simulink model "sim_tcyb_2024_att_ctrl"  (R2020a)
settings: Solver=ode4  StartTime=0.0  StopTime=30.0  FixedStep=0.01  RelTol=1e-3
values from neighbouring files (symbols this model uses):
  c1_diff_sigma_bar_w = diag([12; 12; 12])    [init_tcyb_2024_att_ctrl.m]
  c1_diff_ui = diag([25; 30; 20])    [init_tcyb_2024_att_ctrl.m]
  c2_diff_sigma_bar_w = diag([12; 12; 12])    [init_tcyb_2024_att_ctrl.m]
  c2_diff_ui = diag([50; 50; 10])    [init_tcyb_2024_att_ctrl.m]
  c3_diff_sigma_bar_w = diag([15; 15; 15])    [init_tcyb_2024_att_ctrl.m]
  c3_diff_ui = diag([15; 15; 10])    [init_tcyb_2024_att_ctrl.m]
  dw_aa_t = 0.2 * ones(3, 5) + ( 1.0 - 0.2 ) * rand(3, 5)    [init_tcyb_2024_att_ctrl.m]
  dw_ff_t = [ 0.4 * ones(1, 5) + ( 1.0 - 0.4 ) * rand(1, 5);                      0.4 * ones(1, 5) + ( 1.0 - 0.4 ) * rand(1, 5);                      0.2 * ones(1, 5) + ( 0.6 - 0.2 ) * rand(1, 5) ]    [init_tcyb_2024_att_ctrl.m]
  dw_phi_t = ( - pi / 2 ) * ones(3, 5) + ( pi / 2 - ( - pi / 2 ) ) * rand(3, 5)    [init_tcyb_2024_att_ctrl.m]
  dwci_init = zeros(3,NF)    [init_tcyb_2024_att_ctrl.m]
  h1w = diag([20.0; 20.0; 20.0])    [init_tcyb_2024_att_ctrl.m]
  h2w = diag([30.0; 35.0; 35.0])    [init_tcyb_2024_att_ctrl.m]
  h3w = diag([30.0; 25.0; 30.0])    [init_tcyb_2024_att_ctrl.m]
  Ji = zeros(3,3,NF)    [init_tcyb_2024_att_ctrl.m]
  ksg = diag([10.0, 10.0, 8.0])    [init_tcyb_2024_att_ctrl.m]
  kw = diag([10.0, 10.0, 8.0])    [init_tcyb_2024_att_ctrl.m]
  l1 = diag([5.0, 5.0, 4.0])    [init_tcyb_2024_att_ctrl.m]
  l2 = diag([5.0, 5.0, 4.0])    [init_tcyb_2024_att_ctrl.m]
  Lamd_diff_sigma_bar_w = 0.8    [init_tcyb_2024_att_ctrl.m]
  Lamd_diff_ui = 0.8    [init_tcyb_2024_att_ctrl.m]
  mu = diag([10.0, 10.0, 10.0, 8.0, 8.0, 8.0])    [init_tcyb_2024_att_ctrl.m]
  mu_d_w = 100    [init_tcyb_2024_att_ctrl.m]
  pos0 = zeros(3, 1)    [init_tcyb_2024_att_ctrl.m]
  PZ0 = P0(3)    [init_tcyb_2024_att_ctrl.m]
  PZ1 = 10    [init_tcyb_2024_att_ctrl.m]
  R0 = 4    [init_tcyb_2024_att_ctrl.m]
  R1 = 8    [init_tcyb_2024_att_ctrl.m]
  Rei_init = zeros(3,3,NF)    [init_tcyb_2024_att_ctrl.m]
  Ri_init = zeros(3,3,NF)    [init_tcyb_2024_att_ctrl.m]
  Rx2 = 10    [init_tcyb_2024_att_ctrl.m]
  Ry2 = 6    [init_tcyb_2024_att_ctrl.m]
  Rz2 = 4    [init_tcyb_2024_att_ctrl.m]
  sgei_init = zeros(3,NF)    [init_tcyb_2024_att_ctrl.m]
  sgi_init = zeros(3,NF)    [init_tcyb_2024_att_ctrl.m]
  T0 = 0    [init_tcyb_2024_att_ctrl.m]
  T1 = tseq1    (= 10)    [init_tcyb_2024_att_ctrl.m]
  T2 = tseq1 + tseq12 + tseq2    (= 30)    [init_tcyb_2024_att_ctrl.m]
  ui_init = zeros(3,NF)    [init_tcyb_2024_att_ctrl.m]
  V_Phi_Rei_init = zeros(3,NF)    [init_tcyb_2024_att_ctrl.m]
  vel0 = zeros(3, 1)    [init_tcyb_2024_att_ctrl.m]
  wci_init = zeros(3,NF)    [init_tcyb_2024_att_ctrl.m]
  wei_init = zeros(3,NF)    [init_tcyb_2024_att_ctrl.m]
  zeta_diff_sigma_bar_w = 0.3    [init_tcyb_2024_att_ctrl.m]
  zeta_diff_ui = 0.05    [init_tcyb_2024_att_ctrl.m]
undefined symbols (not defined in the file or in its folder): cal_frac_squ, p_alfaw1, p_alfaw2, q_alfaw1, q_alfaw2, wi_init
(part 1 of 5)
settings Model: Creator=zzy  LastModifiedBy=Hershey.A
settings DataIOCC: ReturnWorkspaceOutputs=off
settings DebuggingCC: ArithmeticOperatorsInVariantConditions=warning
settings SFSimCC: SimUseLocalCustomCode=off  CustomCodeUndefinedFunction=UseInterfaceOnly
settings RTWCC: RTWUseLocalCustomCode=off

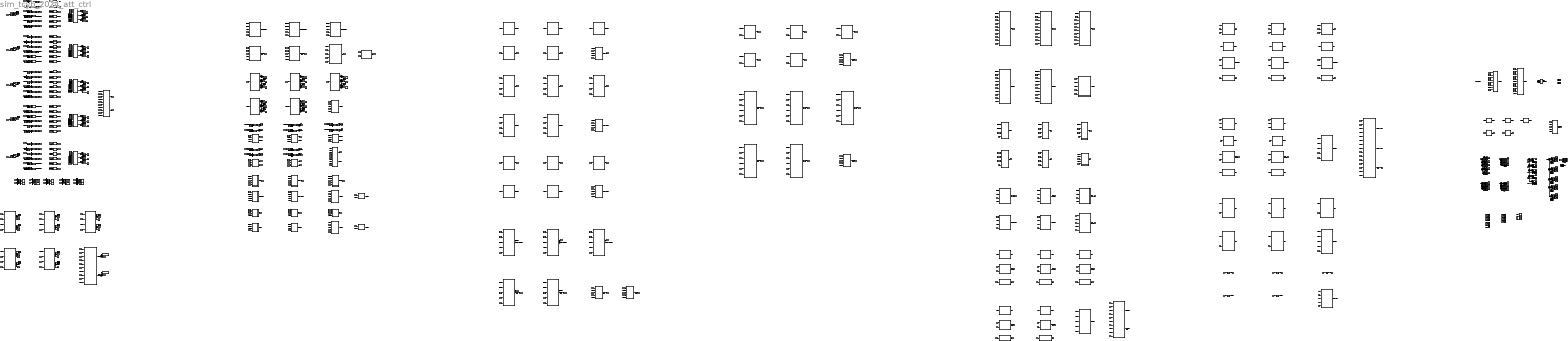
== system sim_tcyb_2024_att_ctrl ==
  Abs{,1..29} (30 alike) : Abs
  Add{,1..2,4..6,8..10,12,14..16,18..19} (15 alike) : Sum
  Add{3,7,11,13,17} (5 alike) : Sum  Inputs=+-
  Clock : Clock
  Constant{,78,96,128,156} (5 alike) : Constant  Value=0
  Constant{1,4,7,10,13} (5 alike) : Constant  Value=l1
  Constant{51,54,59,61,63,79,82,87,89,91,97,100,105,107,109,114,119,121,123,139,142,147,149,151,157} (25 alike) : Constant
  Constant{52..53,55,62,74..75,80..81,83,90,92..93,98..99,101,108,110..111,115,122,124..125,140..141,143,150,152..153,158..159} (30 alike) : Constant  Value=3
  Constant{56,76,84,94,102,112,116,126,144,154} (10 alike) : Constant  Value=2
  Constant{57,85,103,117,145} (5 alike) : Constant  Value=c1_diff_ui
  Constant{58,86,104,118,146} (5 alike) : Constant  Value=c2_diff_ui
  Constant{60,88,106,120,148} (5 alike) : Constant  Value=c3_diff_ui
  Constant{2,5,8,11,14} (5 alike) : Constant  Value=l2
  Constant{77,95,113,127,155} (5 alike) : Constant  Value=Lamd_diff_ui
  Constant{3,6,9,12,15,22,24,26,28,30} (10 alike) : Constant  Value=ksg
  Constant129 : Constant  Value=R0
  Constant130 : Constant  Value=R1
  Constant131 : Constant  Value=T0
  Constant132 : Constant  Value=Rz2
  Constant133 : Constant  Value=Ry2
  Constant134 : Constant  Value=Rx2
  Constant{16..20} (5 alike) : Constant  Value=mu
  Constant{160..174} (15 alike) : Constant  Value=zeta_diff_ui
  Constant{31,175..179,191,201,223,232,235..237,239,241,243} (16 alike) : Constant  Value=Ji
  Constant{190,212,230..231,233..234,238,240,242,244} (10 alike) : Constant  Value=h3w
  Constant{192,194,199,205,210} (5 alike) : Constant  Value=p_alfaw1
  Constant{193,195,200,206,211} (5 alike) : Constant  Value=mu_d_w
  Constant{196,202,207,213,216} (5 alike) : Constant  Value=q_alfaw1
  Constant{197,203,208,214,217} (5 alike) : Constant  Value=p_alfaw2
  Constant{198,204,209,215,218} (5 alike) : Constant  Value=q_alfaw2
  Constant{21,23,25,27,29} (5 alike) : Constant  Value=kw
  Constant{219,221,224,226,228} (5 alike) : Constant  Value=h1w
  Constant{220,222,225,227,229} (5 alike) : Constant  Value=h2w
  Constant32 : Constant  Value=T1
  Constant{557,561,564,567,570} (5 alike) : Constant  Value=dw_aa_t
  Constant{558,562,565,568,572} (5 alike) : Constant  Value=dw_ff_t
  Constant{559,563,566,569,573} (5 alike) : Constant  Value=dw_phi_t
  Constant64 : Constant  Value=T2
  Constant65 : Constant  Value=R0
  Constant66 : Constant  Value=R1
  Constant67 : Constant  Value=Rx2
  Constant68 : Constant  Value=Ry2
  Constant69 : Constant  Value=Rz2
  Constant70 : Constant  Value=T2
  Constant71 : Constant  Value=T1
  Constant72 : Constant  Value=PZ0
  Constant73 : Constant  Value=PZ1
  Demux{,1..20,22..37,42..56,62..76,82..91} (77 alike) : Demux  Outputs=3
  Demux{57..61} (5 alike) : Demux  Outputs=6
  Display{1..15,22..36,38,42..53,59..60,66..70,76..80,91..117} (82 alike) : Display
  E_sgei agent 1 : MATLAB Function  TreatAsAtomicUnit=on
  E_sgei agent 2 : MATLAB Function  TreatAsAtomicUnit=on
  E_sgei agent 3 : MATLAB Function  TreatAsAtomicUnit=on
  E_sgei agent 4 : MATLAB Function  TreatAsAtomicUnit=on
  E_sgei agent 5 : MATLAB Function  TreatAsAtomicUnit=on
  E_sgi agent 1 : MATLAB Function  TreatAsAtomicUnit=on
  E_sgi agent 2 : MATLAB Function  TreatAsAtomicUnit=on
  E_sgi agent 3 : MATLAB Function  TreatAsAtomicUnit=on
  E_sgi agent 4 : MATLAB Function  TreatAsAtomicUnit=on
  E_sgi agent 5 : MATLAB Function  TreatAsAtomicUnit=on
  Integrator{1..15,34..38,46..50} (25 alike) : Integrator  InitialCondition=zeros(3,1)
  Integrator16 : Integrator  InitialCondition=sgi_init(:,2)
  Integrator17 : Integrator  InitialCondition=V_Phi_Rei_init(:,2)
  Integrator18 : Integrator  InitialCondition=sgi_init(:,3)
  Integrator19 : Integrator  InitialCondition=V_Phi_Rei_init(:,3)
  Integrator20 : Integrator  InitialCondition=V_Phi_Rei_init(:,1)
  Integrator21 : Integrator  InitialCondition=wi_init(:,1)
  Integrator22 : Integrator  InitialCondition=wi_init(:,2)
  Integrator23 : Integrator  InitialCondition=wi_init(:,3)
  Integrator24 : Integrator  InitialCondition=wi_init(:,4)
  Integrator25 : Integrator  InitialCondition=wi_init(:,5)
  Integrator26 : Integrator  InitialCondition=sgi_init(:,1)
  Integrator27 : Integrator  InitialCondition=sgi_init(:,4)
  Integrator28 : Integrator  InitialCondition=sgi_init(:,5)
  Integrator29 : Integrator  InitialCondition=sgei_init(:,2)
  Integrator30 : Integrator  InitialCondition=sgei_init(:,3)
  Integrator31 : Integrator  InitialCondition=sgei_init(:,1)
  Integrator32 : Integrator  InitialCondition=sgei_init(:,4)
  Integrator33 : Integrator  InitialCondition=sgei_init(:,5)
  Integrator{39..41,43,45} (5 alike) : Integrator  InitialCondition=zeros(6,1)
  Integrator42 : Integrator  InitialCondition=V_Phi_Rei_init(:,4)
  Integrator44 : Integrator  InitialCondition=V_Phi_Rei_init(:,5)
  Interpreted MATLAB Function{,6..34,50..59} (40 alike) : MATLABFcn  MATLABFcn=cal_frac_squ(u(1:3),u(4),u(5))
  Memory : Memory  InitialCondition=ui_init
  Memory10 : Memory  InitialCondition=zeros(3,3,5)
  Memory11 : Memory  InitialCondition=zeros(3,6,5)
  Memory12 : Memory  InitialCondition=V_Phi_Rei_init
  Memory13 : Memory  InitialCondition=zeros(3,5)
  Memory14 : Memory  InitialCondition=wci_init
  Memory15 : Memory  InitialCondition=dwci_init
  Memory16 : Memory  InitialCondition=zeros(3,6,5)
  Memory17 : Memory  InitialCondition=zeros(3,5)
  Memory18 : Memory  InitialCondition=zeros(3,5)
  Memory19 : Memory  InitialCondition=zeros(3,6,5)
  Memory20 : Memory  InitialCondition=zeros(6,5)
  Memory21 : Memory  InitialCondition=zeros(3,3,5)
  Memory3 : Memory  InitialCondition=sgi_init
  Memory4 : Memory  InitialCondition=Ri_init
  Memory5 : Memory  InitialCondition=wi_init
  Memory6 : Memory  InitialCondition=wei_init
  Memory7 : Memory  InitialCondition=sgei_init
  Memory8 : Memory  InitialCondition=Rei_init
  Memory9 : Memory  InitialCondition=zeros(3,3,5)
  Mux{,1..5,36..65,76..99} (60 alike) : Mux  Inputs=2
  Mux{6..35,66..75} (40 alike) : Mux  Inputs=3
  Mux100 : Mux  Inputs=6
  Product{,1..9} (10 alike) : Product
  Scope{,1..39} (40 alike) : Scope  NumInputPorts=3
  Step : Step  Time=T1+0.01  SampleTime=0
  To Workspace : ToWorkspace  VariableName=wci  SampleTime=-1
  To Workspace1 : ToWorkspace  VariableName=V_Phi_Rei  SampleTime=-1
  To Workspace10 : ToWorkspace  VariableName=dwi_tilt  SampleTime=-1
  To Workspace11 : ToWorkspace  VariableName=thetai  SampleTime=-1
  To Workspace12 : ToWorkspace  VariableName=sigma_bar_w_hat  SampleTime=-1
  To Workspace13 : ToWorkspace  VariableName=wei  SampleTime=-1
  To Workspace14 : ToWorkspace  VariableName=sigma_w  SampleTime=-1
  To Workspace15 : ToWorkspace  VariableName=sigma_bar_w  SampleTime=-1
  To Workspace19 : ToWorkspace  VariableName=sgei  SampleTime=-1
  To Workspace2 : ToWorkspace  VariableName=wi  SampleTime=-1
  To Workspace20 : ToWorkspace  VariableName=sgi  SampleTime=-1
  To Workspace3 : ToWorkspace  VariableName=u0  SampleTime=-1
  To Workspace4 : ToWorkspace  VariableName=eta0  SampleTime=-1
  To Workspace5 : ToWorkspace  VariableName=ksi0  SampleTime=-1
  To Workspace6 : ToWorkspace  VariableName=zetai  SampleTime=-1
  To Workspace7 : ToWorkspace  VariableName=thetai_hat  SampleTime=-1
  To Workspace8 : ToWorkspace  VariableName=dwi  SampleTime=-1
  To Workspace9 : ToWorkspace  VariableName=dwi_hat  SampleTime=-1
  cal Fi agent 1 : MATLAB Function  TreatAsAtomicUnit=on
  cal Fi agent 2 : MATLAB Function  TreatAsAtomicUnit=on
  cal Fi agent 3 : MATLAB Function  TreatAsAtomicUnit=on
  cal Fi agent 4 : MATLAB Function  TreatAsAtomicUnit=on
  cal Fi agent 5 : MATLAB Function  TreatAsAtomicUnit=on
  cal Gamma_Fi agent 1 : MATLAB Function  TreatAsAtomicUnit=on
  cal Gamma_Fi agent 2 : MATLAB Function  TreatAsAtomicUnit=on
  cal Gamma_Fi agent 3 : MATLAB Function  TreatAsAtomicUnit=on
  cal Gamma_Fi agent 4 : MATLAB Function  TreatAsAtomicUnit=on
  cal Gamma_Fi agent 5 : MATLAB Function  TreatAsAtomicUnit=on
  cal Gamma_Fi_min_dzetai agent 1 : MATLAB Function  TreatAsAtomicUnit=on
  cal Gamma_Fi_min_dzetai agent 2 : MATLAB Function  TreatAsAtomicUnit=on
  cal Gamma_Fi_min_dzetai agent 3 : MATLAB Function  TreatAsAtomicUnit=on
  cal Gamma_Fi_min_dzetai agent 4 : MATLAB Function  TreatAsAtomicUnit=on
  cal Gamma_Fi_min_dzetai agent 5 : MATLAB Function  TreatAsAtomicUnit=on
  cal Gamma_wi agent 1 : MATLAB Function  TreatAsAtomicUnit=on
  cal Gamma_wi agent 2 : MATLAB Function  TreatAsAtomicUnit=on
  cal Gamma_wi agent 3 : MATLAB Function  TreatAsAtomicUnit=on
  cal Gamma_wi agent 4 : MATLAB Function  TreatAsAtomicUnit=on
  cal Gamma_wi agent 5 : MATLAB Function  TreatAsAtomicUnit=on
  cal Rci agent 1 : MATLAB Function  TreatAsAtomicUnit=on
  cal Rci agent 2 : MATLAB Function  TreatAsAtomicUnit=on
  cal Rci agent 3 : MATLAB Function  TreatAsAtomicUnit=on
  cal Rci agent 4 : MATLAB Function  TreatAsAtomicUnit=on
  cal Rci agent 5 : MATLAB Function  TreatAsAtomicUnit=on
  cal Rei agent 1 : MATLAB Function  TreatAsAtomicUnit=on
  cal Rei agent 2 : MATLAB Function  TreatAsAtomicUnit=on
  cal Rei agent 3 : MATLAB Function  TreatAsAtomicUnit=on
  cal Rei agent 4 : MATLAB Function  TreatAsAtomicUnit=on
  cal Rei agent 5 : MATLAB Function  TreatAsAtomicUnit=on
  cal Ri agent 1 : MATLAB Function  TreatAsAtomicUnit=on
  cal Ri agent 2 : MATLAB Function  TreatAsAtomicUnit=on
  cal Ri agent 3 : MATLAB Function  TreatAsAtomicUnit=on
  cal Ri agent 4 : MATLAB Function  TreatAsAtomicUnit=on
  cal Ri agent 5 : MATLAB Function  TreatAsAtomicUnit=on
  cal abs 11 : MATLAB Function  TreatAsAtomicUnit=on
  cal abs 12 : MATLAB Function  TreatAsAtomicUnit=on
  cal abs 13 : MATLAB Function  TreatAsAtomicUnit=on
  cal abs 14 : MATLAB Function  TreatAsAtomicUnit=on
  cal abs 15 : MATLAB Function  TreatAsAtomicUnit=on
  cal abs 16 : MATLAB Function  TreatAsAtomicUnit=on
  cal abs 17 : MATLAB Function  TreatAsAtomicUnit=on
  cal abs 18 : MATLAB Function  TreatAsAtomicUnit=on
  cal abs 19 : MATLAB Function  TreatAsAtomicUnit=on
  cal abs 20 : MATLAB Function  TreatAsAtomicUnit=on
  cal combine sigma_bar_w_tilt : MATLAB Function  TreatAsAtomicUnit=on
  cal d_sigma_w agent 1 : MATLAB Function  TreatAsAtomicUnit=on
  cal d_sigma_w agent 2 : MATLAB Function  TreatAsAtomicUnit=on
  cal d_sigma_w agent 3 : MATLAB Function  TreatAsAtomicUnit=on
  cal d_sigma_w agent 4 : MATLAB Function  TreatAsAtomicUnit=on
  cal d_sigma_w agent 5 : MATLAB Function  TreatAsAtomicUnit=on
  cal d_theta_hat : MATLAB Function  TreatAsAtomicUnit=on
  cal d_theta_hat1 : MATLAB Function  TreatAsAtomicUnit=on
  cal d_theta_hat2 : MATLAB Function  TreatAsAtomicUnit=on
  cal d_theta_hat3 : MATLAB Function  TreatAsAtomicUnit=on
  cal d_theta_hat4 : MATLAB Function  TreatAsAtomicUnit=on
  cal differentiator d_sigma_bar_w_hat agent 1 : Subsystem
  cal differentiator d_sigma_bar_w_hat agent 2 : Subsystem
  cal differentiator d_sigma_bar_w_hat agent 3 : Subsystem
  cal differentiator d_sigma_bar_w_hat agent 4 : Subsystem
  cal differentiator d_sigma_bar_w_hat agent 5 : Subsystem
  cal dw_hat agent 1 : MATLAB Function  TreatAsAtomicUnit=on
  cal dw_hat agent 2 : MATLAB Function  TreatAsAtomicUnit=on
  cal dw_hat agent 3 : MATLAB Function  TreatAsAtomicUnit=on
  cal dw_hat agent 4 : MATLAB Function  TreatAsAtomicUnit=on
  cal dw_hat agent 5 : MATLAB Function  TreatAsAtomicUnit=on
  cal error dw_tilt : MATLAB Function  TreatAsAtomicUnit=on
  cal sig : MATLAB Function  TreatAsAtomicUnit=on
  cal sig1 : MATLAB Function  TreatAsAtomicUnit=on
  cal sig10 : MATLAB Function  TreatAsAtomicUnit=on
  cal sig11 : MATLAB Function  TreatAsAtomicUnit=on
  cal sig12 : MATLAB Function  TreatAsAtomicUnit=on
  cal sig13 : MATLAB Function  TreatAsAtomicUnit=on
  cal sig14 : MATLAB Function  TreatAsAtomicUnit=on
  cal sig15 : MATLAB Function  TreatAsAtomicUnit=on
  cal sig16 : MATLAB Function  TreatAsAtomicUnit=on
  cal sig17 : MATLAB Function  TreatAsAtomicUnit=on
  cal sig18 : MATLAB Function  TreatAsAtomicUnit=on
  cal sig19 : MATLAB Function  TreatAsAtomicUnit=on
  cal sig2 : MATLAB Function  TreatAsAtomicUnit=on
  cal sig20 : MATLAB Function  TreatAsAtomicUnit=on
  cal sig21 : MATLAB Function  TreatAsAtomicUnit=on
  cal sig22 : MATLAB Function  TreatAsAtomicUnit=on
  cal sig23 : MATLAB Function  TreatAsAtomicUnit=on
  cal sig24 : MATLAB Function  TreatAsAtomicUnit=on
  cal sig25 : MATLAB Function  TreatAsAtomicUnit=on
  cal sig26 : MATLAB Function  TreatAsAtomicUnit=on
  cal sig27 : MATLAB Function  TreatAsAtomicUnit=on
  cal sig28 : MATLAB Function  TreatAsAtomicUnit=on
  cal sig29 : MATLAB Function  TreatAsAtomicUnit=on
  cal sig3 : MATLAB Function  TreatAsAtomicUnit=on
  cal sig4 : MATLAB Function  TreatAsAtomicUnit=on
  cal sig5 : MATLAB Function  TreatAsAtomicUnit=on
  cal sig6 : MATLAB Function  TreatAsAtomicUnit=on
  cal sig7 : MATLAB Function  TreatAsAtomicUnit=on
  cal sig8 : MATLAB Function  TreatAsAtomicUnit=on
  cal sig9 : MATLAB Function  TreatAsAtomicUnit=on
  cal sigma_bar_w_hat agent 1 : MATLAB Function  TreatAsAtomicUnit=on
  cal sigma_bar_w_hat agent 2 : MATLAB Function  TreatAsAtomicUnit=on
  cal sigma_bar_w_hat agent 3 : MATLAB Function  TreatAsAtomicUnit=on
  cal sigma_bar_w_hat agent 4 : MATLAB Function  TreatAsAtomicUnit=on
  cal sigma_bar_w_hat agent 5 : MATLAB Function  TreatAsAtomicUnit=on
  cal sigma_w_bar : MATLAB Function  TreatAsAtomicUnit=on
  cal taui agent 1 : MATLAB Function  TreatAsAtomicUnit=on
  cal taui agent 2 : MATLAB Function  TreatAsAtomicUnit=on
  cal taui agent 3 : MATLAB Function  TreatAsAtomicUnit=on
  cal taui agent 4 : MATLAB Function  TreatAsAtomicUnit=on
  cal taui agent 5 : MATLAB Function  TreatAsAtomicUnit=on
  cal theta_sigma_bar_w_tilt agent 1 : MATLAB Function  TreatAsAtomicUnit=on
  cal theta_sigma_bar_w_tilt agent 2 : MATLAB Function  TreatAsAtomicUnit=on
  cal theta_sigma_bar_w_tilt agent 3 : MATLAB Function  TreatAsAtomicUnit=on
  cal theta_sigma_bar_w_tilt agent 4 : MATLAB Function  TreatAsAtomicUnit=on
  cal theta_sigma_bar_w_tilt agent 5 : MATLAB Function  TreatAsAtomicUnit=on
  cal thetai_hat agent 1 : MATLAB Function  TreatAsAtomicUnit=on
  cal thetai_hat agent 2 : MATLAB Function  TreatAsAtomicUnit=on
  cal thetai_hat agent 3 : MATLAB Function  TreatAsAtomicUnit=on
  cal thetai_hat agent 4 : MATLAB Function  TreatAsAtomicUnit=on
  cal thetai_hat agent 5 : MATLAB Function  TreatAsAtomicUnit=on
  cal wci dwci agent 1 : MATLAB Function  TreatAsAtomicUnit=on
  cal wci dwci agent 2 : MATLAB Function  TreatAsAtomicUnit=on
  cal wci dwci agent 3 : MATLAB Function  TreatAsAtomicUnit=on
  cal wci dwci agent 4 : MATLAB Function  TreatAsAtomicUnit=on
  cal wci dwci agent 5 : MATLAB Function  TreatAsAtomicUnit=on
  cal wei agent 1 : MATLAB Function  TreatAsAtomicUnit=on
  cal wei agent 2 : MATLAB Function  TreatAsAtomicUnit=on
  cal wei agent 3 : MATLAB Function  TreatAsAtomicUnit=on
  cal wei agent 4 : MATLAB Function  TreatAsAtomicUnit=on
  cal wei agent 5 : MATLAB Function  TreatAsAtomicUnit=on
  cal zetai agent 1 : MATLAB Function  TreatAsAtomicUnit=on
  cal zetai agent 2 : MATLAB Function  TreatAsAtomicUnit=on
  cal zetai agent 3 : MATLAB Function  TreatAsAtomicUnit=on
  cal zetai agent 4 : MATLAB Function  TreatAsAtomicUnit=on
  cal zetai agent 5 : MATLAB Function  TreatAsAtomicUnit=on
  choose ksi_est_err 11 : MATLAB Function  TreatAsAtomicUnit=on
  choose ksi_est_err 12 : MATLAB Function  TreatAsAtomicUnit=on
  choose ksi_est_err 13 : MATLAB Function  TreatAsAtomicUnit=on
  choose ksi_est_err 14 : MATLAB Function  TreatAsAtomicUnit=on
  choose ksi_est_err 15 : MATLAB Function  TreatAsAtomicUnit=on
  choose ksi_est_err 16 : MATLAB Function  TreatAsAtomicUnit=on
  choose ksi_est_err 17 : MATLAB Function  TreatAsAtomicUnit=on
  choose ksi_est_err 18 : MATLAB Function  TreatAsAtomicUnit=on
  choose ksi_est_err 19 : MATLAB Function  TreatAsAtomicUnit=on
  choose ksi_est_err 20 : MATLAB Function  TreatAsAtomicUnit=on
  choose ui agent 1 : MATLAB Function  TreatAsAtomicUnit=on
  choose ui agent 2 : MATLAB Function  TreatAsAtomicUnit=on
  choose ui agent 3 : MATLAB Function  TreatAsAtomicUnit=on
  choose ui agent 4 : MATLAB Function  TreatAsAtomicUnit=on
  choose ui agent 5 : MATLAB Function  TreatAsAtomicUnit=on
  combine E_sgi_vec : MATLAB Function  TreatAsAtomicUnit=on
  combine E_sgi_vec1 : MATLAB Function  TreatAsAtomicUnit=on
  combine Fi_vec : MATLAB Function  TreatAsAtomicUnit=on
  combine Gamma_Fi_min_dzetai : MATLAB Function  TreatAsAtomicUnit=on
  combine Gamma_Fi_vec : MATLAB Function  TreatAsAtomicUnit=on
  combine Gamma_wi_vec : MATLAB Function  TreatAsAtomicUnit=on
  combine Qci Rci1 : MATLAB Function  TreatAsAtomicUnit=on
  combine Rci : MATLAB Function  TreatAsAtomicUnit=on
  combine d_sigma_bar_v_est : MATLAB Function  TreatAsAtomicUnit=on
  combine d_zetai_vec : MATLAB Function  TreatAsAtomicUnit=on
  combine duihat d2uihat : MATLAB Function  TreatAsAtomicUnit=on
  combine dw_hat : MATLAB Function  TreatAsAtomicUnit=on
  combine dwi : MATLAB Function  TreatAsAtomicUnit=on
  combine norminal formation control input : MATLAB Function  TreatAsAtomicUnit=on
  combine sgi Ri : MATLAB Function  TreatAsAtomicUnit=on
  combine sigma_bar_w_hat : MATLAB Function  TreatAsAtomicUnit=on
  combine sigma_w : MATLAB Function  TreatAsAtomicUnit=on
  combine tau : MATLAB Function  TreatAsAtomicUnit=on
  combine tau1 : MATLAB Function  TreatAsAtomicUnit=on
  combine theta_sigma_bar_w_tilt : MATLAB Function  TreatAsAtomicUnit=on
  combine thetai_hat : MATLAB Function  TreatAsAtomicUnit=on
  combine wci dwci : MATLAB Function  TreatAsAtomicUnit=on
  combine wei Qei Rei : MATLAB Function  TreatAsAtomicUnit=on
  combine zetai_vec : MATLAB Function  TreatAsAtomicUnit=on
  control input generator agent 1 : MATLAB Function  TreatAsAtomicUnit=on
  control input generator agent 2 : MATLAB Function  TreatAsAtomicUnit=on
  control input generator agent 3 : MATLAB Function  TreatAsAtomicUnit=on
  control input generator agent 4 : MATLAB Function  TreatAsAtomicUnit=on
  control input generator agent 5 : MATLAB Function  TreatAsAtomicUnit=on
  d2_sigma_bar_w_est_{1..5} (5 alike) : Scope  NumInputPorts=3
  d2_ui_hat_node_{1..5} (5 alike) : Scope  NumInputPorts=3
  d_sigma_bar_w_est_{1..5} (5 alike) : Scope  NumInputPorts=3
  d_ui_hat_node_{1..5} (5 alike) : Scope  NumInputPorts=3
  depart Ji_1_1 : MATLAB Function  TreatAsAtomicUnit=on
  depart Ji_1_2 : MATLAB Function  TreatAsAtomicUnit=on
  depart Ji_1_3 : MATLAB Function  TreatAsAtomicUnit=on
  depart Ji_2_2 : MATLAB Function  TreatAsAtomicUnit=on
  depart Ji_2_3 : MATLAB Function  TreatAsAtomicUnit=on
  depart Ji_3_3 : MATLAB Function  TreatAsAtomicUnit=on
  depart V_Phi_Re1 : MATLAB Function  TreatAsAtomicUnit=on
  depart V_Phi_Re2 : MATLAB Function  TreatAsAtomicUnit=on
  depart V_Phi_Re3 : MATLAB Function  TreatAsAtomicUnit=on
  depart V_Phi_Re4 : MATLAB Function  TreatAsAtomicUnit=on
  depart V_Phi_Re5 : MATLAB Function  TreatAsAtomicUnit=on
  depart sge1 : MATLAB Function  TreatAsAtomicUnit=on
  depart sge2 : MATLAB Function  TreatAsAtomicUnit=on
  depart sge3 : MATLAB Function  TreatAsAtomicUnit=on
  depart sge4 : MATLAB Function  TreatAsAtomicUnit=on
  depart sge5 : MATLAB Function  TreatAsAtomicUnit=on
  depart theta_hat_1 : MATLAB Function  TreatAsAtomicUnit=on
  depart theta_hat_2 : MATLAB Function  TreatAsAtomicUnit=on
  depart theta_hat_3 : MATLAB Function  TreatAsAtomicUnit=on
  depart theta_hat_4 : MATLAB Function  TreatAsAtomicUnit=on
  depart theta_hat_5 : MATLAB Function  TreatAsAtomicUnit=on
  depart wc1 : MATLAB Function  TreatAsAtomicUnit=on
  depart wc2 : MATLAB Function  TreatAsAtomicUnit=on
  depart wc3 : MATLAB Function  TreatAsAtomicUnit=on
  depart wc4 : MATLAB Function  TreatAsAtomicUnit=on
  depart wc5 : MATLAB Function  TreatAsAtomicUnit=on
  depart we1 : MATLAB Function  TreatAsAtomicUnit=on
  depart we2 : MATLAB Function  TreatAsAtomicUnit=on
  depart we3 : MATLAB Function  TreatAsAtomicUnit=on
  depart we4 : MATLAB Function  TreatAsAtomicUnit=on
  depart we5 : MATLAB Function  TreatAsAtomicUnit=on
  depart zetai_1 : MATLAB Function  TreatAsAtomicUnit=on
  depart zetai_2 : MATLAB Function  TreatAsAtomicUnit=on
  depart zetai_3 : MATLAB Function  TreatAsAtomicUnit=on
  depart zetai_4 : MATLAB Function  TreatAsAtomicUnit=on
  depart zetai_5 : MATLAB Function  TreatAsAtomicUnit=on
  dsgei dynam agent 1 : MATLAB Function  TreatAsAtomicUnit=on
  dsgei dynam agent 2 : MATLAB Function  TreatAsAtomicUnit=on
  dsgei dynam agent 3 : MATLAB Function  TreatAsAtomicUnit=on
  dsgei dynam agent 4 : MATLAB Function  TreatAsAtomicUnit=on
  dsgei dynam agent 5 : MATLAB Function  TreatAsAtomicUnit=on
  dwci_node_{1..5} (5 alike) : Scope  NumInputPorts=3
  eta_0 : Scope  NumInputPorts=3
  generate angular rate disturbance agent 1 : MATLAB Function  TreatAsAtomicUnit=on
  generate angular rate disturbance agent 2 : MATLAB Function  TreatAsAtomicUnit=on
  generate angular rate disturbance agent 3 : MATLAB Function  TreatAsAtomicUnit=on
  generate angular rate disturbance agent 4 : MATLAB Function  TreatAsAtomicUnit=on
  generate angular rate disturbance agent 5 : MATLAB Function  TreatAsAtomicUnit=on
  ksi_0 : Scope  NumInputPorts=3
  leader control input : MATLAB Function  TreatAsAtomicUnit=on
  leader eta0 Integrator : Integrator  ExternalReset=rising  InitialConditionSource=external  InitialCondition=vel0
  leader ksi0 Integrator : Integrator  InitialCondition=pos0
  process velocity : MATLAB Function  TreatAsAtomicUnit=on
  sgi dynam agent 1 : MATLAB Function  TreatAsAtomicUnit=on
  sgi dynam agent 2 : MATLAB Function  TreatAsAtomicUnit=on
  sgi dynam agent 3 : MATLAB Function  TreatAsAtomicUnit=on
  sgi dynam agent 4 : MATLAB Function  TreatAsAtomicUnit=on
  sgi dynam agent 5 : MATLAB Function  TreatAsAtomicUnit=on
  sigma_bar_w_hat Integrator {1..5} (5 alike) : Integrator  InitialCondition=zeros(3,1)
  trans to column10 : MATLAB Function  TreatAsAtomicUnit=on
  trans to column11 : MATLAB Function  TreatAsAtomicUnit=on
  trans to column12 : MATLAB Function  TreatAsAtomicUnit=on
  trans to column13 : MATLAB Function  TreatAsAtomicUnit=on
  trans to column14 : MATLAB Function  TreatAsAtomicUnit=on
  trans to column15 : MATLAB Function  TreatAsAtomicUnit=on
  trans to column16 : MATLAB Function  TreatAsAtomicUnit=on
  trans to column17 : MATLAB Function  TreatAsAtomicUnit=on
  trans to column18 : MATLAB Function  TreatAsAtomicUnit=on
  trans to column19 : MATLAB Function  TreatAsAtomicUnit=on
  trans to column20 : MATLAB Function  TreatAsAtomicUnit=on
  trans to column21 : MATLAB Function  TreatAsAtomicUnit=on
  trans to column22 : MATLAB Function  TreatAsAtomicUnit=on
  trans to column23 : MATLAB Function  TreatAsAtomicUnit=on
  trans to column24 : MATLAB Function  TreatAsAtomicUnit=on
  trans to column25 : MATLAB Function  TreatAsAtomicUnit=on
  trans to column26 : MATLAB Function  TreatAsAtomicUnit=on
  trans to column27 : MATLAB Function  TreatAsAtomicUnit=on
  trans to column28 : MATLAB Function  TreatAsAtomicUnit=on
  trans to column29 : MATLAB Function  TreatAsAtomicUnit=on
  trans to column30 : MATLAB Function  TreatAsAtomicUnit=on
  trans to column31 : MATLAB Function  TreatAsAtomicUnit=on
  trans to column32 : MATLAB Function  TreatAsAtomicUnit=on
  trans to column33 : MATLAB Function  TreatAsAtomicUnit=on
  trans to column34 : MATLAB Function  TreatAsAtomicUnit=on
  trans to column5 : MATLAB Function  TreatAsAtomicUnit=on
  trans to column51 : MATLAB Function  TreatAsAtomicUnit=on
  trans to column52 : MATLAB Function  TreatAsAtomicUnit=on
  trans to column53 : MATLAB Function  TreatAsAtomicUnit=on
  trans to column54 : MATLAB Function  TreatAsAtomicUnit=on
  trans to column55 : MATLAB Function  TreatAsAtomicUnit=on
  trans to column56 : MATLAB Function  TreatAsAtomicUnit=on
  trans to column57 : MATLAB Function  TreatAsAtomicUnit=on
  trans to column58 : MATLAB Function  TreatAsAtomicUnit=on
  trans to column59 : MATLAB Function  TreatAsAtomicUnit=on
  trans to column6 : MATLAB Function  TreatAsAtomicUnit=on
  trans to column60 : MATLAB Function  TreatAsAtomicUnit=on
  trans to column7 : MATLAB Function  TreatAsAtomicUnit=on
  trans to column8 : MATLAB Function  TreatAsAtomicUnit=on
  trans to column9 : MATLAB Function  TreatAsAtomicUnit=on
  ui_tilt_node_{1..5} (5 alike) : Scope  NumInputPorts=3
  wci_node_{1..5} (5 alike) : Scope  NumInputPorts=3
  wi dynam agent 1 : MATLAB Function  TreatAsAtomicUnit=on
  wi dynam agent 2 : MATLAB Function  TreatAsAtomicUnit=on
  wi dynam agent 3 : MATLAB Function  TreatAsAtomicUnit=on
  wi dynam agent 4 : MATLAB Function  TreatAsAtomicUnit=on
  wi dynam agent 5 : MATLAB Function  TreatAsAtomicUnit=on
  wires:
  [d_ui_hat_node_1] -> cal d_theta_hat/11(dui_hat)
  [ui_sig_3_node_1] -> cal d_theta_hat/7(ui_sig_3)
  cal d_theta_hat/2(d_dui_hat) -> Integrator3/1
  Constant63/1 -> Mux8/2
  Mux10/1 -> Interpreted MATLAB Function9/1
  cal sig5/1(z) -> [ui_sig_5_node_1]
  Interpreted MATLAB Function8/1 -> trans to column8/1(x)
  Interpreted MATLAB Function9/1 -> trans to column9/1(x)
  [ui_squ_3_node_1] -> cal sig2/1(x)
  Constant163/1 -> Product1/2
  [ui_squ_6_node_1] -> cal sig3/1(x)
  [ui_sig_6_node_1] -> cal d_theta_hat/10(ui_sig_6)
  cal d_theta_hat/3(d_d2ui_hat) -> Integrator4/1
  trans to column8/1(y) -> [ui_squ_4_node_1]
  [ui_tilt_node_1] -> cal sig1/2(y)
  [ui_sig_2_node_1] -> cal d_theta_hat/6(ui_sig_2)
  Abs/1 -> Mux7/1
  Constant56/1 -> Mux11/2
  [d2_ui_hat_node_1] -> cal d_theta_hat/12(d2ui_hat)
  cal sig3/1(z) -> [ui_sig_6_node_1]
  Interpreted MATLAB Function7/1 -> trans to column7/1(x)
  Interpreted MATLAB Function/1 -> trans to column6/1(x)
  cal sig4/1(z) -> [ui_sig_4_node_1]
  Product1/1 -> Add2/2
  [ui_tilt_node_1] -> cal sig5/2(y)
  trans to column10/1(y) -> [ui_squ_5_node_1]
  [ui_tilt_node_1] -> cal sig/2(y)
  Interpreted MATLAB Function10/1 -> trans to column10/1(x)
  Mux11/1 -> Interpreted MATLAB Function10/1
  Abs5/1 -> Mux11/1
  Abs3/1 -> Mux9/1
  Constant53/1 -> Add2/1
  Constant/1 -> Mux7/2
  Constant162/1 -> Product/2
  Constant54/1 -> Product1/1
  Constant55/1 -> Mux11/3
  [ui_tilt_node_1] -> Abs4/1
  [ui_sig_4_node_1] -> cal d_theta_hat/8(ui_sig_4)
  [ui_sig_1_node_1] -> cal d_theta_hat/5(ui_sig_1)
  [ui_squ_5_node_1] -> cal sig5/1(x)
  Constant59/1 -> Add/1
  Constant61/1 -> Mux6/3
  Mux7/1 -> Interpreted MATLAB Function/1
  Mux8/1 -> Interpreted MATLAB Function7/1
  Constant161/1 -> Add/2
  [ui_tilt_node_1] -> Abs2/1
  [ui_tilt_node_1] -> Abs1/1
  [ui_tilt_node_1] -> Abs5/1
  Mux6/1 -> Interpreted MATLAB Function6/1
  Interpreted MATLAB Function6/1 -> trans to column5/1(x)
  Add/1 -> Mux6/2
  [ui_squ_4_node_1] -> cal sig4/1(x)
  trans to column9/1(y) -> [ui_squ_6_node_1]
  trans to column7/1(y) -> [ui_squ_3_node_1]
  [ui_tilt_node_1] -> cal sig4/2(y)
  [ui_tilt_node_1] -> cal sig3/2(y)
  Product/1 -> Add1/2
  Constant51/1 -> Mux7/3
  Constant75/1 -> Add1/1
  [ui_tilt_node_1] -> Abs/1
  [ui_tilt_node_1] -> Abs3/1
  Mux9/1 -> Interpreted MATLAB Function8/1
  Abs2/1 -> Mux8/1
  Constant62/1 -> Mux8/3
  trans to column5/1(y) -> [ui_squ_2_node_1]
  cal sig1/1(z) -> [ui_sig_2_node_1]
  Constant52/1 -> Mux10/3
  cal sig/1(z) -> [ui_sig_1_node_1]
  Abs4/1 -> Mux10/1
  cal sig2/1(z) -> [ui_sig_3_node_1]
  Abs1/1 -> Mux6/1
  Constant74/1 -> Mux9/3
  Add2/1 -> Mux10/2
  [ui_sig_5_node_1] -> cal d_theta_hat/9(ui_sig_5)
  Add1/1 -> Mux9/2
  Constant76/1 -> Product/1
  [ui_tilt_node_1] -> cal sig2/2(y)
  [ui_squ_2_node_1] -> cal sig1/1(x)
  [ui_squ_1_node_1] -> cal sig/1(x)
  trans to column6/1(y) -> [ui_squ_1_node_1]
  Constant57/1 -> cal d_theta_hat/1(c1)
  Constant58/1 -> cal d_theta_hat/2(c2)
  Constant60/1 -> cal d_theta_hat/3(c3)
  Constant77/1 -> cal d_theta_hat/4(chi_t)
  Integrator4/1 -> Display24/1, Demux12/1, [d2_ui_hat_node_1]
  cal d_theta_hat/1(d_ui_hat) -> Integrator2/1
  Integrator3/1 -> Demux8/1, Display23/1, [d_ui_hat_node_1]
  Integrator2/1 -> Display22/1, [ui_hat_node_1]
  [ui_hat_node_1] -> Add3/1
  Add3/1 -> Demux2/1, [ui_tilt_node_1]
  [ui_vec] -> choose ui agent 1/1(x)
  choose ui agent 1/1(y) -> Add3/2
  [ui_squ_1_node_2] -> cal sig6/1(x)
  [ui_squ_2_node_2] -> cal sig7/1(x)
  [ui_tilt_node_2] -> cal sig8/2(y)
  Constant94/1 -> Product2/1
  Constant95/1 -> cal d_theta_hat1/4(chi_t)
  Add7/1 -> Demux3/1, [ui_tilt_node_2]
  [ui_hat_node_2] -> Add7/1
  [ui_sig_5_node_2] -> cal d_theta_hat1/9(ui_sig_5)
  Add6/1 -> Mux12/2
  Add5/1 -> Mux17/2
  Constant92/1 -> Mux17/3
  Constant80/1 -> Mux12/3
  cal sig6/1(z) -> [ui_sig_1_node_2]
  trans to column12/1(y) -> [ui_squ_2_node_2]
  cal sig7/1(z) -> [ui_sig_2_node_2]
  cal sig8/1(z) -> [ui_sig_3_node_2]
  Abs7/1 -> Mux14/1
  Abs10/1 -> Mux12/1
  Constant90/1 -> Mux16/3
  [ui_tilt_node_2] -> Abs9/1
  Mux17/1 -> Interpreted MATLAB Function15/1
  choose ui agent 2/1(y) -> Add7/2
  Abs8/1 -> Mux16/1
  Product2/1 -> Add5/2
  [ui_tilt_node_2] -> Abs6/1
  Constant93/1 -> Add5/1
  [ui_tilt_node_2] -> cal sig10/2(y)
  Constant79/1 -> Mux15/3
  trans to column16/1(y) -> [ui_squ_6_node_2]
  Constant88/1 -> cal d_theta_hat1/3(c3)
  Constant85/1 -> cal d_theta_hat1/1(c1)
  Integrator1/1 -> Display25/1, [ui_hat_node_2]
  Integrator6/1 -> Display27/1, Demux13/1, [d2_ui_hat_node_2]
  trans to column15/1(y) -> [ui_squ_4_node_2]
  [ui_sig_6_node_2] -> cal d_theta_hat1/10(ui_sig_6)
  [ui_squ_6_node_2] -> cal sig9/1(x)
  Constant91/1 -> Mux16/2
  [ui_squ_4_node_2] -> cal sig10/1(x)
  [d_ui_hat_node_2] -> cal d_theta_hat1/11(dui_hat)
  Mux14/1 -> Interpreted MATLAB Function13/1
  [ui_tilt_node_2] -> cal sig9/2(y)
  Constant160/1 -> Add4/2
  Constant87/1 -> Add4/1
  Mux12/1 -> Interpreted MATLAB Function16/1
  [ui_squ_5_node_2] -> cal sig11/1(x)
  [ui_sig_1_node_2] -> cal d_theta_hat1/5(ui_sig_1)
  [ui_tilt_node_2] -> Abs8/1
  [ui_sig_4_node_2] -> cal d_theta_hat1/8(ui_sig_4)
  [ui_tilt_node_2] -> Abs10/1
  cal d_theta_hat1/2(d_dui_hat) -> Integrator5/1
  Constant89/1 -> Mux14/3
  Constant83/1 -> Mux13/3
  Constant82/1 -> Product3/1
  Abs9/1 -> Mux17/1
  Interpreted MATLAB Function11/1 -> trans to column13/1(x)
  Mux16/1 -> Interpreted MATLAB Function14/1
  trans to column13/1(y) -> [ui_squ_1_node_2]
  Interpreted MATLAB Function16/1 -> trans to column16/1(x)
  Interpreted MATLAB Function12/1 -> trans to column11/1(x)
  Constant81/1 -> Add6/1
  Abs11/1 -> Mux13/1
  cal sig10/1(z) -> [ui_sig_4_node_2]
  [ui_tilt_node_2] -> cal sig6/2(y)
  Constant78/1 -> Mux15/2
  Interpreted MATLAB Function14/1 -> trans to column14/1(x)
  Constant164/1 -> Product2/2
  [ui_vec] -> choose ui agent 2/1(x)
  [d2_ui_hat_node_2] -> cal d_theta_hat1/12(d2ui_hat)
  Add4/1 -> Mux14/2
  trans to column11/1(y) -> [ui_squ_5_node_2]
  cal d_theta_hat1/1(d_ui_hat) -> Integrator1/1
  Constant165/1 -> Product3/2
  cal sig9/1(z) -> [ui_sig_6_node_2]
  Abs6/1 -> Mux15/1
  [ui_tilt_node_2] -> Abs7/1
  Interpreted MATLAB Function15/1 -> trans to column15/1(x)
  cal d_theta_hat1/3(d_d2ui_hat) -> Integrator6/1
  [ui_sig_2_node_2] -> cal d_theta_hat1/6(ui_sig_2)
  Product3/1 -> Add6/2
  Mux15/1 -> Interpreted MATLAB Function11/1
  [ui_tilt_node_2] -> Abs11/1
  [ui_tilt_node_2] -> cal sig11/2(y)
  Interpreted MATLAB Function13/1 -> trans to column12/1(x)
  [ui_tilt_node_2] -> cal sig7/2(y)
  Constant84/1 -> Mux13/2
  Mux13/1 -> Interpreted MATLAB Function12/1
  [ui_sig_3_node_2] -> cal d_theta_hat1/7(ui_sig_3)
  trans to column14/1(y) -> [ui_squ_3_node_2]
  Constant86/1 -> cal d_theta_hat1/2(c2)
  cal sig11/1(z) -> [ui_sig_5_node_2]
  [ui_squ_3_node_2] -> cal sig8/1(x)
  [ui_squ_4_node_3] -> cal sig12/1(x)
  Constant109/1 -> Mux22/2
  [ui_squ_6_node_3] -> cal sig17/1(x)
  [ui_sig_6_node_3] -> cal d_theta_hat2/10(ui_sig_6)
  trans to column21/1(y) -> [ui_squ_4_node_3]
  Integrator9/1 -> Display30/1, Demux14/1, [d2_ui_hat_node_3]
  Integrator8/1 -> Display29/1, Demux7/1, [d_ui_hat_node_3]
  Integrator7/1 -> Display28/1, [ui_hat_node_3]
  Constant103/1 -> cal d_theta_hat2/1(c1)
  Constant106/1 -> cal d_theta_hat2/3(c3)
  [ui_tilt_node_3] -> Abs14/1
  trans to column22/1(y) -> [ui_squ_6_node_3]
  Constant97/1 -> Mux21/3
  Product4/1 -> Add9/2
  [ui_tilt_node_3] -> cal sig12/2(y)
  Constant111/1 -> Add9/1
  Abs12/1 -> Mux18/1
  cal sig16/1(z) -> [ui_sig_3_node_3]
  Constant108/1 -> Mux22/3
  [ui_tilt_node_3] -> Abs17/1
  Abs15/1 -> Mux20/1
  Abs16/1 -> Mux22/1
  choose ui agent 3/1(y) -> Add11/2
  Mux23/1 -> Interpreted MATLAB Function21/1
  cal sig15/1(z) -> [ui_sig_2_node_3]
  trans to column18/1(y) -> [ui_squ_2_node_3]
  cal sig14/1(z) -> [ui_sig_1_node_3]
  Constant98/1 -> Mux18/3
  Add11/1 -> Demux4/1, [ui_tilt_node_3]
  Constant113/1 -> cal d_theta_hat2/4(chi_t)
  Constant112/1 -> Product4/1
  Constant110/1 -> Mux23/3
  Add9/1 -> Mux23/2
  [ui_sig_5_node_3] -> cal d_theta_hat2/9(ui_sig_5)
  [ui_hat_node_3] -> Add11/1
  Add10/1 -> Mux18/2
  [ui_tilt_node_3] -> cal sig16/2(y)
  [ui_sig_1_node_3] -> cal d_theta_hat2/5(ui_sig_1)
  [ui_sig_4_node_3] -> cal d_theta_hat2/8(ui_sig_4)
  Mux18/1 -> Interpreted MATLAB Function22/1
  [ui_tilt_node_3] -> cal sig17/2(y)
  [ui_squ_5_node_3] -> cal sig13/1(x)
  Mux20/1 -> Interpreted MATLAB Function19/1
  Interpreted MATLAB Function18/1 -> trans to column17/1(x)
  [ui_tilt_node_3] -> Abs12/1
  Mux22/1 -> Interpreted MATLAB Function20/1
  Interpreted MATLAB Function17/1 -> trans to column19/1(x)
  Abs17/1 -> Mux23/1
  cal sig17/1(z) -> [ui_sig_6_node_3]
  Abs13/1 -> Mux19/1
  cal d_theta_hat2/1(d_ui_hat) -> Integrator7/1
  trans to column19/1(y) -> [ui_squ_1_node_3]
  trans to column17/1(y) -> [ui_squ_5_node_3]
  [d_ui_hat_node_3] -> cal d_theta_hat2/11(dui_hat)
  [d2_ui_hat_node_3] -> cal d_theta_hat2/12(d2ui_hat)
  Interpreted MATLAB Function22/1 -> trans to column22/1(x)
  Interpreted MATLAB Function20/1 -> trans to column20/1(x)
  cal d_theta_hat2/2(d_dui_hat) -> Integrator8/1
  Constant167/1 -> Product4/2
  Constant101/1 -> Mux19/3
  Constant105/1 -> Add8/1
  Constant96/1 -> Mux21/2
  [ui_tilt_node_3] -> cal sig14/2(y)
  cal sig12/1(z) -> [ui_sig_4_node_3]
  Constant168/1 -> Product5/2
  cal sig13/1(z) -> [ui_sig_5_node_3]
  [ui_squ_3_node_3] -> cal sig16/1(x)
  [ui_sig_3_node_3] -> cal d_theta_hat2/7(ui_sig_3)
  Mux19/1 -> Interpreted MATLAB Function18/1
  Constant104/1 -> cal d_theta_hat2/2(c2)
  Constant102/1 -> Mux19/2
  trans to column20/1(y) -> [ui_squ_3_node_3]
  [ui_tilt_node_3] -> Abs16/1
  Interpreted MATLAB Function19/1 -> trans to column18/1(x)
  [ui_tilt_node_3] -> cal sig15/2(y)
  Constant166/1 -> Add8/2
  [ui_tilt_node_3] -> Abs13/1
  [ui_tilt_node_3] -> cal sig13/2(y)
  [ui_squ_1_node_3] -> cal sig14/1(x)
  [ui_sig_2_node_3] -> cal d_theta_hat2/6(ui_sig_2)
  [ui_tilt_node_3] -> Abs15/1
  Interpreted MATLAB Function21/1 -> trans to column21/1(x)
  [ui_vec] -> choose ui agent 3/1(x)
  Constant99/1 -> Add10/1
  cal d_theta_hat2/3(d_d2ui_hat) -> Integrator9/1
  Abs14/1 -> Mux21/1
  Constant107/1 -> Mux20/3
  Product5/1 -> Add10/2
  [ui_squ_2_node_3] -> cal sig15/1(x)
  Add8/1 -> Mux20/2
  Constant100/1 -> Product5/1
  Mux21/1 -> Interpreted MATLAB Function17/1
  [ui_vec] -> choose ui agent 4/1(x)
  [ui_sig_2_node_4] -> cal d_theta_hat3/6(ui_sig_2)
  [ui_tilt_node_4] -> cal sig19/2(y)
  [ui_squ_1_node_4] -> cal sig20/1(x)
  [ui_tilt_node_4] -> Abs19/1
  trans to column26/1(y) -> [ui_squ_3_node_4]
  Constant169/1 -> Add14/2
  Interpreted MATLAB Function25/1 -> trans to column24/1(x)
  [ui_tilt_node_4] -> cal sig21/2(y)
  [ui_tilt_node_4] -> Abs22/1
  [ui_squ_3_node_4] -> cal sig22/1(x)
  [ui_sig_3_node_4] -> cal d_theta_hat3/7(ui_sig_3)
  Constant116/1 -> Mux25/2
  Mux25/1 -> Interpreted MATLAB Function24/1
  cal sig19/1(z) -> [ui_sig_5_node_4]
  Constant128/1 -> Mux27/2
  [ui_tilt_node_4] -> cal sig20/2(y)
  Constant171/1 -> Product7/2
  cal sig18/1(z) -> [ui_sig_4_node_4]
  Constant119/1 -> Add14/1
  Constant115/1 -> Mux25/3
  Constant170/1 -> Product6/2
  cal d_theta_hat3/2(d_dui_hat) -> Integrator11/1
  Interpreted MATLAB Function26/1 -> trans to column26/1(x)
  Interpreted MATLAB Function28/1 -> trans to column28/1(x)
  cal d_theta_hat3/1(d_ui_hat) -> Integrator10/1
  [d2_ui_hat_node_4] -> cal d_theta_hat3/12(d2ui_hat)
  [d_ui_hat_node_4] -> cal d_theta_hat3/11(dui_hat)
  trans to column23/1(y) -> [ui_squ_5_node_4]
  Constant118/1 -> cal d_theta_hat3/2(c2)
  Interpreted MATLAB Function24/1 -> trans to column23/1(x)
  Abs23/1 -> Mux29/1
  [ui_squ_5_node_4] -> cal sig19/1(x)
  [ui_tilt_node_4] -> Abs18/1
  [ui_tilt_node_4] -> cal sig23/2(y)
  Mux24/1 -> Interpreted MATLAB Function28/1
  Add15/1 -> Mux29/2
  Add12/1 -> Mux24/2
  Interpreted MATLAB Function23/1 -> trans to column25/1(x)
  Abs19/1 -> Mux25/1
  Constant124/1 -> Mux29/3
  trans to column24/1(y) -> [ui_squ_2_node_4]
  Constant140/1 -> Mux24/3
  Mux29/1 -> Interpreted MATLAB Function27/1
  cal sig21/1(z) -> [ui_sig_2_node_4]
  Abs21/1 -> Mux26/1
  Abs18/1 -> Mux24/1
  [ui_tilt_node_4] -> Abs23/1
  [ui_sig_5_node_4] -> cal d_theta_hat3/9(ui_sig_5)
  Constant122/1 -> Mux28/3
  Constant125/1 -> Add15/1
  cal sig22/1(z) -> [ui_sig_3_node_4]
  Abs22/1 -> Mux28/1
  [ui_tilt_node_4] -> cal sig18/2(y)
  Constant117/1 -> cal d_theta_hat3/1(c1)
  Constant120/1 -> cal d_theta_hat3/3(c3)
  cal sig20/1(z) -> [ui_sig_1_node_4]
  trans to column28/1(y) -> [ui_squ_6_node_4]
  Integrator10/1 -> [ui_hat_node_4], Display31/1
  [ui_tilt_node_4] -> Abs20/1
  Product6/1 -> Add15/2
  trans to column25/1(y) -> [ui_squ_1_node_4]
  [ui_squ_6_node_4] -> cal sig23/1(x)
  Integrator11/1 -> Display32/1, Demux10/1, [d_ui_hat_node_4]
  trans to column27/1(y) -> [ui_squ_4_node_4]
  [ui_hat_node_4] -> Add13/1
  Constant126/1 -> Product6/1
  Integrator12/1 -> Display33/1, Demux15/1, [d2_ui_hat_node_4]
  Constant139/1 -> Mux27/3
  [ui_squ_4_node_4] -> cal sig18/1(x)
  Constant127/1 -> cal d_theta_hat3/4(chi_t)
  Constant123/1 -> Mux28/2
  [ui_tilt_node_4] -> Abs21/1
  Interpreted MATLAB Function27/1 -> trans to column27/1(x)
  choose ui agent 4/1(y) -> Add13/2
  Add13/1 -> Demux5/1, [ui_tilt_node_4]
  [ui_sig_6_node_4] -> cal d_theta_hat3/10(ui_sig_6)
  [ui_squ_2_node_4] -> cal sig21/1(x)
  Constant121/1 -> Mux26/3
  Product7/1 -> Add12/2
  Add14/1 -> Mux26/2
  Abs20/1 -> Mux27/1
  cal d_theta_hat3/3(d_d2ui_hat) -> Integrator12/1
  [ui_sig_4_node_4] -> cal d_theta_hat3/8(ui_sig_4)
  cal sig23/1(z) -> [ui_sig_6_node_4]
  Constant141/1 -> Add12/1
  [ui_sig_1_node_4] -> cal d_theta_hat3/5(ui_sig_1)
  Mux26/1 -> Interpreted MATLAB Function25/1
  Mux27/1 -> Interpreted MATLAB Function23/1
  Constant114/1 -> Product7/1
  [ui_tilt_node_4] -> cal sig22/2(y)
  Mux28/1 -> Interpreted MATLAB Function26/1
  Constant155/1 -> cal d_theta_hat4/4(chi_t)
  [ui_squ_2_node_5] -> cal sig27/1(x)
  Interpreted MATLAB Function33/1 -> trans to column33/1(x)
  choose ui agent 5/1(y) -> Add17/2
  Constant151/1 -> Mux34/2
  [ui_sig_6_node_5] -> cal d_theta_hat4/10(ui_sig_6)
  [ui_squ_4_node_5] -> cal sig24/1(x)
  Integrator15/1 -> Display36/1, Demux16/1, [d2_ui_hat_node_5]
  Constant154/1 -> Product8/1
  [ui_hat_node_5] -> Add17/1
  trans to column31/1(y) -> [ui_squ_1_node_5]
  Constant157/1 -> Mux33/3
  Integrator14/1 -> Display35/1, Demux11/1, [d_ui_hat_node_5]
  Constant145/1 -> cal d_theta_hat4/1(c1)
  Abs28/1 -> Mux34/1
  trans to column34/1(y) -> [ui_squ_6_node_5]
  [ui_tilt_node_5] -> cal sig24/2(y)
  Integrator13/1 -> Display34/1, [ui_hat_node_5]
  cal sig26/1(z) -> [ui_sig_1_node_5]
  Constant148/1 -> cal d_theta_hat4/3(c3)
  Mux35/1 -> Interpreted MATLAB Function33/1
  [ui_tilt_node_5] -> Abs29/1
  [ui_sig_5_node_5] -> cal d_theta_hat4/9(ui_sig_5)
  cal sig27/1(z) -> [ui_sig_2_node_5]
  Constant153/1 -> Add19/1
  Constant150/1 -> Mux34/3
  Abs24/1 -> Mux30/1
  Mux30/1 -> Interpreted MATLAB Function34/1
  Interpreted MATLAB Function29/1 -> trans to column31/1(x)
  trans to column30/1(y) -> [ui_squ_2_node_5]
  Abs27/1 -> Mux32/1
  Add16/1 -> Mux30/2
  Add19/1 -> Mux35/2
  Constant158/1 -> Mux30/3
  [ui_tilt_node_5] -> Abs24/1
  Abs29/1 -> Mux35/1
  Constant146/1 -> cal d_theta_hat4/2(c2)
  Interpreted MATLAB Function30/1 -> trans to column29/1(x)
  [ui_squ_5_node_5] -> cal sig25/1(x)
  trans to column29/1(y) -> [ui_squ_5_node_5]
  Product8/1 -> Add19/2
  Constant143/1 -> Mux31/3
  Add17/1 -> Demux6/1, [ui_tilt_node_5]
  cal d_theta_hat4/2(d_dui_hat) -> Integrator14/1
  Abs25/1 -> Mux31/1
  cal d_theta_hat4/1(d_ui_hat) -> Integrator13/1
  Interpreted MATLAB Function34/1 -> trans to column34/1(x)
  Interpreted MATLAB Function32/1 -> trans to column32/1(x)
  [ui_squ_6_node_5] -> cal sig29/1(x)
  Constant173/1 -> Product8/2
  cal sig24/1(z) -> [ui_sig_4_node_5]
  Constant156/1 -> Mux33/2
  [ui_tilt_node_5] -> cal sig26/2(y)
  trans to column33/1(y) -> [ui_squ_4_node_5]
  Constant147/1 -> Add18/1
  cal sig25/1(z) -> [ui_sig_5_node_5]
  [ui_sig_3_node_5] -> cal d_theta_hat4/7(ui_sig_3)
  Mux31/1 -> Interpreted MATLAB Function30/1
  [ui_tilt_node_5] -> Abs25/1
  [ui_tilt_node_5] -> Abs28/1
  Constant144/1 -> Mux31/2
  [ui_tilt_node_5] -> cal sig25/2(y)
  [ui_tilt_node_5] -> Abs27/1
  Interpreted MATLAB Function31/1 -> trans to column30/1(x)
  [d_ui_hat_node_5] -> cal d_theta_hat4/11(dui_hat)
  Constant172/1 -> Add18/2
  [ui_tilt_node_5] -> Abs26/1
  trans to column32/1(y) -> [ui_squ_3_node_5]
  [ui_squ_3_node_5] -> cal sig28/1(x)
  Constant152/1 -> Mux35/3
  [ui_sig_2_node_5] -> cal d_theta_hat4/6(ui_sig_2)
  [ui_vec] -> choose ui agent 5/1(x)
  [ui_squ_1_node_5] -> cal sig26/1(x)
  [ui_tilt_node_5] -> cal sig28/2(y)
  cal sig28/1(z) -> [ui_sig_3_node_5]
  Constant142/1 -> Product9/1
  Constant159/1 -> Add16/1
  [ui_sig_1_node_5] -> cal d_theta_hat4/5(ui_sig_1)
  Mux32/1 -> Interpreted MATLAB Function31/1
  Mux33/1 -> Interpreted MATLAB Function29/1
  Mux34/1 -> Interpreted MATLAB Function32/1
  Product9/1 -> Add16/2
  cal sig29/1(z) -> [ui_sig_6_node_5]
  Add18/1 -> Mux32/2
  Constant174/1 -> Product9/2
  Constant149/1 -> Mux32/3
  [d2_ui_hat_node_5] -> cal d_theta_hat4/12(d2ui_hat)
  Abs26/1 -> Mux33/1
  cal d_theta_hat4/3(d_d2ui_hat) -> Integrator15/1
  [ui_tilt_node_5] -> cal sig27/2(y)
  [ui_tilt_node_5] -> cal sig29/2(y)
  [ui_sig_4_node_5] -> cal d_theta_hat4/8(ui_sig_4)
  combine duihat d2uihat/2(d2uihat_vec) -> [d2uihat_vec]
  combine duihat d2uihat/1(duihat_vec) -> [duihat_vec]
  [d_ui_hat_node_1] -> combine duihat d2uihat/1(d_ui_hat_node_1)
  [d_ui_hat_node_2] -> combine duihat d2uihat/2(d_ui_hat_node_2)
  [d_ui_hat_node_3] -> combine duihat d2uihat/3(d_ui_hat_node_3)
  [d_ui_hat_node_4] -> combine duihat d2uihat/4(d_ui_hat_node_4)
  [d_ui_hat_node_5] -> combine duihat d2uihat/5(d_ui_hat_node_5)
  [d2_ui_hat_node_1] -> combine duihat d2uihat/6(d2_ui_hat_node_1)
  [d2_ui_hat_node_2] -> combine duihat d2uihat/7(d2_ui_hat_node_2)
  [d2_ui_hat_node_3] -> combine duihat d2uihat/8(d2_ui_hat_node_3)
  [d2_ui_hat_node_4] -> combine duihat d2uihat/9(d2_ui_hat_node_4)
  [d2_ui_hat_node_5] -> combine duihat d2uihat/10(d2_ui_hat_node_5)
  [ui_vec] -> cal wci dwci agent 1/1(ui_vec)
  [duihat_vec] -> cal wci dwci agent 1/2(duihat_vec)
  [d2uihat_vec] -> cal wci dwci agent 1/3(d2uihat_vec)
  [Rci_vec] -> cal wci dwci agent 1/4(Rci_mat)
  cal wci dwci agent 1/2(dwci) -> Display45/1, Demux18/1, [dwci_node_1]
  [ui_vec] -> cal wci dwci agent 2/1(ui_vec)
  cal wci dwci agent 2/2(dwci) -> Display47/1, Demux20/1, [dwci_node_2]
  cal wci dwci agent 2/1(wci) -> Demux19/1, Display46/1, [wci_node_2]
  [d2uihat_vec] -> cal wci dwci agent 2/3(d2uihat_vec)
  [Rci_vec] -> cal wci dwci agent 2/4(Rci_mat)
  [duihat_vec] -> cal wci dwci agent 2/2(duihat_vec)
  [Rci_vec] -> cal wci dwci agent 3/4(Rci_mat)
  cal wci dwci agent 3/1(wci) -> Display48/1, Demux42/1, [wci_node_3]
  [ui_vec] -> cal wci dwci agent 3/1(ui_vec)
  [duihat_vec] -> cal wci dwci agent 3/2(duihat_vec)
  [d2uihat_vec] -> cal wci dwci agent 3/3(d2uihat_vec)
  [Rci_vec] -> cal wci dwci agent 4/4(Rci_mat)
  [ui_vec] -> cal wci dwci agent 4/1(ui_vec)
  [duihat_vec] -> cal wci dwci agent 4/2(duihat_vec)
  cal wci dwci agent 4/1(wci) -> Display50/1, Demux44/1, [wci_node_4]
  cal wci dwci agent 4/2(dwci) -> Display51/1, Demux45/1, [dwci_node_4]
  [d2uihat_vec] -> cal wci dwci agent 4/3(d2uihat_vec)
  cal wci dwci agent 5/1(wci) -> Display52/1, Demux46/1, [wci_node_5]
  [d2uihat_vec] -> cal wci dwci agent 5/3(d2uihat_vec)
  [Rci_vec] -> cal wci dwci agent 5/4(Rci_mat)
  [duihat_vec] -> cal wci dwci agent 5/2(duihat_vec)
  cal wci dwci agent 5/2(dwci) -> Display53/1, Demux47/1, [dwci_node_5]
  [ui_vec] -> cal wci dwci agent 5/1(ui_vec)
  [wci_node_1] -> combine wci dwci/1(wci_node_1)
  [wci_node_2] -> combine wci dwci/2(wci_node_2)
  [wci_node_3] -> combine wci dwci/3(wci_node_3)
  [wci_node_4] -> combine wci dwci/4(wci_node_4)
  [wci_node_5] -> combine wci dwci/5(wci_node_5)
  [dwci_node_1] -> combine wci dwci/6(dwci_node_1)
  [dwci_node_2] -> combine wci dwci/7(dwci_node_2)
  [dwci_node_3] -> combine wci dwci/8(dwci_node_3)
  [dwci_node_4] -> combine wci dwci/9(dwci_node_4)
  [dwci_node_5] -> combine wci dwci/10(dwci_node_5)
  Demux2/2 -> ui_tilt_node_1/2
  Demux2/3 -> ui_tilt_node_1/3
  Demux2/1 -> ui_tilt_node_1/1
  Demux3/3 -> ui_tilt_node_2/3
  Demux3/1 -> ui_tilt_node_2/1
  Demux3/2 -> ui_tilt_node_2/2
  Demux4/3 -> ui_tilt_node_3/3
  Demux4/1 -> ui_tilt_node_3/1
  Demux4/2 -> ui_tilt_node_3/2
  Demux5/3 -> ui_tilt_node_4/3
  Demux5/1 -> ui_tilt_node_4/1
  Demux5/2 -> ui_tilt_node_4/2
  Demux6/3 -> ui_tilt_node_5/3
  Demux6/1 -> ui_tilt_node_5/1
  Demux6/2 -> ui_tilt_node_5/2
  Demux7/3 -> d_ui_hat_node_3/3
  Demux7/1 -> d_ui_hat_node_3/1
  Demux7/2 -> d_ui_hat_node_3/2
  Demux8/2 -> d_ui_hat_node_1/2
  Demux8/1 -> d_ui_hat_node_1/1
  Demux8/3 -> d_ui_hat_node_1/3
  Demux9/2 -> d_ui_hat_node_2/2
  Demux9/1 -> d_ui_hat_node_2/1
  Demux9/3 -> d_ui_hat_node_2/3
  Integrator5/1 -> Display26/1, [d_ui_hat_node_2], Demux9/1
  Demux10/2 -> d_ui_hat_node_4/2
  Demux10/1 -> d_ui_hat_node_4/1
  Demux10/3 -> d_ui_hat_node_4/3
  Demux11/2 -> d_ui_hat_node_5/2
  Demux11/1 -> d_ui_hat_node_5/1
  Demux11/3 -> d_ui_hat_node_5/3
  Demux12/2 -> d2_ui_hat_node_1/2
  Demux12/1 -> d2_ui_hat_node_1/1
  Demux12/3 -> d2_ui_hat_node_1/3
  Demux13/3 -> d2_ui_hat_node_2/3
  Demux13/2 -> d2_ui_hat_node_2/2
  Demux13/1 -> d2_ui_hat_node_2/1
  Demux14/3 -> d2_ui_hat_node_3/3
  Demux14/2 -> d2_ui_hat_node_3/2
  Demux14/1 -> d2_ui_hat_node_3/1
  Demux15/3 -> d2_ui_hat_node_4/3
  Demux15/2 -> d2_ui_hat_node_4/2
  Demux15/1 -> d2_ui_hat_node_4/1
  Demux16/3 -> d2_ui_hat_node_5/3
  Demux16/2 -> d2_ui_hat_node_5/2
  Demux16/1 -> d2_ui_hat_node_5/1
  Demux17/3 -> wci_node_1/3
  Demux17/1 -> wci_node_1/1
  Demux17/2 -> wci_node_1/2
  Demux18/1 -> dwci_node_1/1
  Demux18/2 -> dwci_node_1/2
  Demux18/3 -> dwci_node_1/3
  Demux19/2 -> wci_node_2/2
  Demux19/1 -> wci_node_2/1
  Demux19/3 -> wci_node_2/3
  Demux20/2 -> dwci_node_2/2
  Demux20/1 -> dwci_node_2/1
  Demux20/3 -> dwci_node_2/3
  Demux42/3 -> wci_node_3/3
  Demux42/2 -> wci_node_3/2
  Demux42/1 -> wci_node_3/1
  Demux43/3 -> dwci_node_3/3
  Demux43/2 -> dwci_node_3/2
  Demux43/1 -> dwci_node_3/1
  Demux44/3 -> wci_node_4/3
  Demux44/2 -> wci_node_4/2
  Demux44/1 -> wci_node_4/1
  Demux45/3 -> dwci_node_4/3
  Demux45/1 -> dwci_node_4/1
  Demux45/2 -> dwci_node_4/2
  Demux46/3 -> wci_node_5/3
  Demux46/1 -> wci_node_5/1
  Demux46/2 -> wci_node_5/2
  Demux47/3 -> dwci_node_5/3
  Demux47/1 -> dwci_node_5/1
  Demux47/2 -> dwci_node_5/2
  cal wci dwci agent 1/1(wci) -> Display44/1, Demux17/1, [wci_node_1]
  cal wci dwci agent 3/2(dwci) -> [dwci_node_3], Display49/1, Demux43/1
  combine wci dwci/1(wci_vec) -> Memory14/1
  combine wci dwci/2(dwci_vec) -> Memory15/1
  [ui_hat_node_4] -> Demux53/1
  Demux48/3 -> Mux43/2
  Demux56/2 -> Mux54/2
  Demux54/3 -> Mux49/2
  Mux50/1 -> Scope14/1
  Demux48/2 -> Mux42/2
  Demux49/1 -> Mux48/1
  Mux54/1 -> Scope15/2
  Demux50/1 -> Mux48/2
  Demux55/2 -> Mux54/1
  Mux49/1 -> Scope14/3
  Demux51/2 -> Mux47/1
  [ui_5] -> Demux56/1
  [ui_hat_node_5] -> Demux55/1
  Mux53/1 -> Scope15/1
  [ui_4] -> Demux54/1
  Demux52/2 -> Mux47/2
  Mux52/1 -> Scope15/3
  Demux53/1 -> Mux50/1
  Demux55/1 -> Mux53/1
  Demux54/1 -> Mux50/2
  Demux54/2 -> Mux51/2
  Mux45/1 -> Scope13/3
  [ui_3] -> Demux52/1
  Demux52/3 -> Mux45/2
  Demux51/3 -> Mux45/1
  [ui_1] -> Demux48/1
  Demux55/3 -> Mux52/1
  Demux50/2 -> Mux55/2
  Mux46/1 -> Scope13/1
  Mux42/1 -> Scope2/2
  Demux52/1 -> Mux46/2
  Demux56/1 -> Mux53/2
  [ui_hat_node_3] -> Demux51/1
  [ui_hat_node_2] -> Demux49/1
  Demux/2 -> Mux42/1
  Mux48/1 -> Scope1/1
  Demux49/3 -> Mux44/1
  Demux49/2 -> Mux55/1
  Mux44/1 -> Scope1/3
  Mux47/1 -> Scope13/2
  Demux/3 -> Mux43/1
  [ui_2] -> Demux50/1
  Mux43/1 -> Scope2/3
  Demux53/3 -> Mux49/1
  Mux51/1 -> Scope14/2
  Mux55/1 -> Scope1/2
  Demux56/3 -> Mux52/2
  Mux41/1 -> Scope2/1
  Demux53/2 -> Mux51/1
  Demux/1 -> Mux41/1
  [ui_hat_node_1] -> Demux/1
  Demux50/3 -> Mux44/2
  Demux51/1 -> Mux46/1
  Demux48/1 -> Mux41/2
  [tau_1] -> combine tau/1(tau_1)
  [tau_2] -> combine tau/2(tau_2)
  [tau_3] -> combine tau/3(tau_3)
  [tau_4] -> combine tau/4(tau_4)
  [tau_5] -> combine tau/5(tau_5)
  combine tau/1(taui_vec) -> [taui_vec]
  [wi_vec] -> wi dynam agent 1/2(wi_vec)
  Constant175/1 -> wi dynam agent 1/1(Ji)
  [taui_vec] -> wi dynam agent 1/3(taui_vec)
  wi dynam agent 1/1(dwi_1) -> Integrator21/1
  [taui_vec] -> wi dynam agent 2/3(taui_vec)
  [wi_vec] -> wi dynam agent 2/2(wi_vec)
  wi dynam agent 2/1(dwi_2) -> Integrator22/1
  Constant176/1 -> wi dynam agent 2/1(Ji)
  Constant177/1 -> wi dynam agent 3/1(Ji)
  [wi_vec] -> wi dynam agent 3/2(wi_vec)
  [taui_vec] -> wi dynam agent 3/3(taui_vec)
  wi dynam agent 3/1(dwi_3) -> Integrator23/1
  [taui_vec] -> wi dynam agent 4/3(taui_vec)
  Constant178/1 -> wi dynam agent 4/1(Ji)
  [wi_vec] -> wi dynam agent 4/2(wi_vec)
  wi dynam agent 4/1(dwi_4) -> Integrator24/1
  [taui_vec] -> wi dynam agent 5/3(taui_vec)
  wi dynam agent 5/1(dwi_5) -> Integrator25/1
  Constant179/1 -> wi dynam agent 5/1(Ji)
  [wi_vec] -> wi dynam agent 5/2(wi_vec)
  [wi_1] -> combine dwi/1(wi_1)
  [wi_2] -> combine dwi/2(wi_2)
  [wi_3] -> combine dwi/3(wi_3)
  [wi_4] -> combine dwi/4(wi_4)
  [wi_5] -> combine dwi/5(wi_5)
  combine dwi/1(wi_vec) -> Memory5/1
  Integrator21/1 -> [wi_1]
  Integrator22/1 -> [wi_2]
  Integrator23/1 -> [wi_3]
  Integrator24/1 -> [wi_4]
  Integrator25/1 -> [wi_5]
  [E_sgi_vec] -> sgi dynam agent 1/1(E_sgi_vec)
  [wi_vec] -> sgi dynam agent 1/2(wi_vec)
  sgi dynam agent 1/1(dsgi_1) -> Integrator26/1
  Integrator26/1 -> [sgi_1]
  [sgi_1] -> combine sgi Ri/1(sgi_1)
  [sgi_2] -> combine sgi Ri/2(sgi_2)
  [sgi_3] -> combine sgi Ri/3(sgi_3)
  [sgi_4] -> combine sgi Ri/4(sgi_4)
  [sgi_5] -> combine sgi Ri/5(sgi_5)
  combine sgi Ri/1(sgi_vec) -> Memory3/1
  [wi_vec] -> cal wei agent 1/1(wi_vec)
  [Rei_vec] -> cal wei agent 1/2(Rei_vec)
  [wci_vec] -> cal wei agent 1/3(wci_vec)
  cal wei agent 1/1(wei_1) -> [wei_1]
  [E_sgei_vec] -> dsgei dynam agent 1/1(E_sgei_vec)
  [wei_vec] -> dsgei dynam agent 1/2(wei_vec)
  Integrator31/1 -> [sgei_1]
  dsgei dynam agent 1/1(dsgei_1) -> Integrator31/1
  [wei_1] -> combine wei Qei Rei/1(wei_1)
  [wei_2] -> combine wei Qei Rei/2(wei_2)
  [wei_3] -> combine wei Qei Rei/3(wei_3)
  [wei_4] -> combine wei Qei Rei/4(wei_4)
  [wei_5] -> combine wei Qei Rei/5(wei_5)
  [sgei_1] -> combine wei Qei Rei/6(sgei_1)
  [sgei_2] -> combine wei Qei Rei/7(sgei_2)
  [sgei_3] -> combine wei Qei Rei/8(sgei_3)
  [sgei_4] -> combine wei Qei Rei/9(sgei_4)
  [sgei_5] -> combine wei Qei Rei/10(sgei_5)
  [Rei_1] -> combine wei Qei Rei/11(Rei_1)
  [Rei_2] -> combine wei Qei Rei/12(Rei_2)
  [Rei_3] -> combine wei Qei Rei/13(Rei_3)
  [Rei_4] -> combine wei Qei Rei/14(Rei_4)
  [Rei_5] -> combine wei Qei Rei/15(Rei_5)
  combine wei Qei Rei/1(wei_vec) -> Memory6/1
  combine wei Qei Rei/2(sgei_vec) -> Memory7/1
  combine wei Qei Rei/3(Rei_vec) -> Memory8/1
  cal Ri agent 1/1(Ri_1) -> [Ri_1]
  [sgi_vec] -> cal Ri agent 1/1(sgi_vec)
  [Ri_1] -> combine sgi Ri/6(Ri_1)
  [Ri_2] -> combine sgi Ri/7(Ri_2)
  [Ri_3] -> combine sgi Ri/8(Ri_3)
  [Ri_4] -> combine sgi Ri/9(Ri_4)
  [Ri_5] -> combine sgi Ri/10(Ri_5)
  combine sgi Ri/2(Ri_vec) -> Memory4/1
  Integrator20/1 -> [V_Phi_Rei_1]
  Integrator17/1 -> [V_Phi_Rei_2]
  Integrator19/1 -> [V_Phi_Rei_3]
  Integrator42/1 -> [V_Phi_Rei_4]
  Integrator44/1 -> [V_Phi_Rei_5]
  combine Qci Rci1/1(V_Phi_Rei_vec) -> Memory12/1
  [V_Phi_Rei_2] -> combine Qci Rci1/2(V_Phi_Rei_2)
  [V_Phi_Rei_3] -> combine Qci Rci1/3(V_Phi_Rei_3)
  [V_Phi_Rei_5] -> combine Qci Rci1/5(V_Phi_Rei_5)
  [V_Phi_Rei_4] -> combine Qci Rci1/4(V_Phi_Rei_4)
  [V_Phi_Rei_1] -> combine Qci Rci1/1(V_Phi_Rei_1)
  [sgei_vec] -> depart sge3/1(x), depart sge5/1(x), depart sge4/1(x), depart sge2/1(x), depart sge1/1(x)
  depart sge1/1(y) -> Display38/1, Demux33/1
  Demux33/1 -> Scope/1
  Demux33/2 -> Scope/2
  Demux33/3 -> Scope/3
  Demux34/1 -> Scope3/1
  Demux34/3 -> Scope3/3
  Demux34/2 -> Scope3/2
  depart sge2/1(y) -> Display42/1, Demux34/1
  Demux35/1 -> Scope4/1
  Demux35/3 -> Scope4/3
  Demux35/2 -> Scope4/2
  depart sge3/1(y) -> Display43/1, Demux35/1
  Demux36/1 -> Scope5/1
  Demux36/3 -> Scope5/3
  Demux36/2 -> Scope5/2
  depart sge4/1(y) -> Display59/1, Demux36/1
  Demux37/1 -> Scope6/1
  Demux37/3 -> Scope6/3
  Demux37/2 -> Scope6/2
  depart sge5/1(y) -> Display60/1, Demux37/1
  Demux62/1 -> Scope17/1
  depart we5/1(y) -> [wei_node_5], Display70/1, Demux66/1
  Demux65/3 -> Scope12/3
  Demux65/2 -> Scope12/2
  Demux66/3 -> Scope16/3
  Demux66/2 -> Scope16/2
  Demux66/1 -> Scope16/1
  Demux65/1 -> Scope12/1
  [wei_vec] -> depart we3/1(x), depart we5/1(x), depart we4/1(x), depart we2/1(x), depart we1/1(x)
  depart we3/1(y) -> [wei_node_3], Display68/1, Demux64/1
  Demux63/1 -> Scope18/1
  depart we2/1(y) -> [wei_node_2], Display67/1, Demux63/1
  Demux63/3 -> Scope18/3
  depart we4/1(y) -> Display69/1, [wei_node_4], Demux65/1
  Demux62/3 -> Scope17/3
  Demux64/1 -> Scope19/1
  Demux64/3 -> Scope19/3
  Demux63/2 -> Scope18/2
  depart we1/1(y) -> [wei_node_1], Display66/1, Demux62/1
  Demux64/2 -> Scope19/2
  Demux62/2 -> Scope17/2
  Demux75/3 -> Scope25/3
  [V_Phi_Rei_vec] -> depart V_Phi_Re3/1(x), depart V_Phi_Re5/1(x), depart V_Phi_Re4/1(x), depart V_Phi_Re2/1(x), depart V_Phi_Re1/1(x)
  depart V_Phi_Re4/1(y) -> Display79/1, Demux75/1
  Demux72/3 -> Scope27/3
  Demux73/2 -> Scope28/2
  Demux74/3 -> Scope29/3
  Demux74/1 -> Scope29/1
  depart V_Phi_Re2/1(y) -> Display77/1, Demux73/1
  depart V_Phi_Re5/1(y) -> Display80/1, Demux76/1
  Demux73/1 -> Scope28/1
  depart V_Phi_Re3/1(y) -> Display78/1, Demux74/1
  Demux73/3 -> Scope28/3
  Demux74/2 -> Scope29/2
  depart V_Phi_Re1/1(y) -> Display76/1, Demux72/1
  Demux72/2 -> Scope27/2
  Demux75/1 -> Scope25/1
  Demux75/2 -> Scope25/2
  Demux72/1 -> Scope27/1
  Demux76/1 -> Scope26/1
  Demux76/3 -> Scope26/3
  Demux76/2 -> Scope26/2
  Memory3/1 -> [sgi_vec]
  Memory4/1 -> [Ri_vec]
  Memory5/1 -> [wi_vec]
  Memory6/1 -> [wei_vec]
  Memory7/1 -> [sgei_vec]
  Memory8/1 -> [Rei_vec]
  Memory12/1 -> [V_Phi_Rei_vec]
  Memory14/1 -> Display100/1, [wci_vec]
  Memory15/1 -> Display101/1, [dwci_vec]
  [wei_1] -> Integrator20/1
  [wei_2] -> Integrator17/1
  [wei_3] -> Integrator19/1
  [wei_4] -> Integrator42/1
  [wei_5] -> Integrator44/1
  depart wc4/1(y) -> Display4/1, Demux26/1
  Demux25/2 -> Scope37/2
  Demux23/2 -> Scope35/2
  depart wc2/1(y) -> Display2/1, Demux24/1
  Demux26/2 -> Scope38/2
  Demux27/2 -> Scope39/2
  Demux27/1 -> Scope39/1
  [wci_vec] -> depart wc3/1(x), depart wc5/1(x), depart wc4/1(x), depart wc2/1(x), depart wc1/1(x)
  Demux27/3 -> Scope39/3
  Demux25/1 -> Scope37/1
  depart wc3/1(y) -> Display3/1, Demux25/1
  Demux26/1 -> Scope38/1
  Demux26/3 -> Scope38/3
  Demux24/3 -> Scope36/3
  depart wc5/1(y) -> Display5/1, Demux27/1
  depart wc1/1(y) -> Display1/1, Demux23/1
  Demux25/3 -> Scope37/3
  Demux23/3 -> Scope35/3
  Demux24/2 -> Scope36/2
  Demux23/1 -> Scope35/1
  Demux24/1 -> Scope36/1
  Constant218/1 -> Mux66/3
  cal abs 11/1(y) -> Mux67/1
  Demux90/2 -> d2_sigma_bar_w_est_5/2
  choose ksi_est_err 17/1(y) -> cal abs 17/1(x)
  sigma_bar_w_hat Integrator 5/1 -> [sigma_bar_w_hat_5]
  Constant213/1 -> Mux74/3
  cal abs 12/1(y) -> Mux66/1
  [dw_hat_5] -> combine dw_hat/5(dw_hat_5)
  cal abs 13/1(y) -> Mux73/1
  [sigma_bar_w_hat_vec] -> cal dw_hat agent 3/4(sigma_bar_w_hat_vec)
  [d_sigma_bar_w_est_5] -> combine d_sigma_bar_v_est/5(d_sigma_bar_w_est_5)
  [sigma_bar_w_hat_5] -> combine sigma_bar_w_hat/5(sigma_bar_w_hat_5)
  [wi_vec] -> cal d_sigma_w agent 4/3(wi_vec)
  Constant220/1 -> cal sigma_bar_w_hat agent 1/2(h2w)
  Demux88/3 -> d2_sigma_bar_w_est_4/3
  Demux85/3 -> d_sigma_bar_w_est_2/3
  [sigma_bar_w_tilt_vec] -> choose ksi_est_err 15/1(x)
  Interpreted MATLAB Function52/1 -> trans to column53/1(x)
  trans to column52/1(y) -> [sigma_bar_w_tilt_squ_1_1], Display98/1
  [wi_vec] -> cal d_sigma_w agent 1/3(wi_vec)
  Constant203/1 -> Mux75/2
  cal theta_sigma_bar_w_tilt agent 1/1(theta_sigma_bar_w_tilt_1_1) -> [theta_sigma_bar_w_tilt_1_1]
  Integrator46/1 -> [sigma_w_1]
  Constant241/1 -> cal dw_hat agent 5/2(Ji)
  [theta_sigma_bar_w_tilt_2_vec] -> cal sigma_bar_w_hat agent 5/4(theta_sigma_bar_w_tilt_2_vec)
  [sigma_bar_w_hat_vec] -> cal dw_hat agent 4/4(sigma_bar_w_hat_vec)
  Constant237/1 -> cal dw_hat agent 1/2(Ji)
  Constant235/1 -> cal dw_hat agent 3/2(Ji)
  trans to column60/1(y) -> [sigma_bar_w_tilt_squ_1_5], Display112/1
  cal dw_hat agent 3/1(dw_hat_3) -> [dw_hat_3]
  [d_sigma_bar_w_vec] -> cal dw_hat agent 3/3(d_sigma_bar_w_vec)
  [d_sigma_bar_w_vec] -> cal dw_hat agent 2/3(d_sigma_bar_w_vec)
  cal sigma_bar_w_hat agent 1/1(d_sigma_bar_w_hat_1) -> sigma_bar_w_hat Integrator 1/1
  cal sigma_bar_w_hat agent 3/1(d_sigma_bar_w_hat_3) -> sigma_bar_w_hat Integrator 3/1
  [d_sigma_bar_w_vec] -> cal sigma_bar_w_hat agent 1/5(d_sigma_bar_w_vec)
  Constant221/1 -> cal sigma_bar_w_hat agent 2/1(h1w)
  [sigma_bar_w_tilt_vec] -> choose ksi_est_err 19/1(x)
  [d_sigma_bar_w_vec] -> cal sigma_bar_w_hat agent 2/5(d_sigma_bar_w_vec)
  [theta_sigma_bar_w_tilt_2_vec] -> cal sigma_bar_w_hat agent 3/4(theta_sigma_bar_w_tilt_2_vec)
  [sigma_bar_w_vec] -> cal differentiator d_sigma_bar_w_hat agent 4/1(x)
  Constant222/1 -> cal sigma_bar_w_hat agent 2/2(h2w)
  [theta_sigma_bar_w_tilt_1_vec] -> cal sigma_bar_w_hat agent 2/3(theta_sigma_bar_w_tilt_1_vec)
  sigma_bar_w_hat Integrator 3/1 -> [sigma_bar_w_hat_3]
  sigma_bar_w_hat Integrator 2/1 -> [sigma_bar_w_hat_2]
  [sigma_bar_w_vec] -> cal combine sigma_bar_w_tilt/1(sigma_bar_w_vec)
  [sigma_bar_w_hat_vec] -> cal dw_hat agent 1/4(sigma_bar_w_hat_vec)
  Constant190/1 -> cal d_sigma_w agent 1/1(h3w)
  combine sigma_w/1(sigma_w_vec) -> [sigma_w_vec]
  cal sigma_bar_w_hat agent 5/1(d_sigma_bar_w_hat_5) -> sigma_bar_w_hat Integrator 5/1
  Constant215/1 -> Mux72/3
  Interpreted MATLAB Function51/1 -> trans to column52/1(x)
  cal dw_hat agent 2/1(dw_hat_2) -> [dw_hat_2]
  cal d_sigma_w agent 3/1(d_sigma_w_3) -> Integrator48/1
  Constant228/1 -> cal sigma_bar_w_hat agent 5/1(h1w)
  [theta_sigma_bar_w_tilt_2_vec] -> cal sigma_bar_w_hat agent 1/4(theta_sigma_bar_w_tilt_2_vec)
  [d_sigma_bar_w_vec] -> cal sigma_bar_w_hat agent 3/5(d_sigma_bar_w_vec)
  [sigma_bar_w_tilt_vec] -> cal theta_sigma_bar_w_tilt agent 5/4(sigma_bar_w_tilt_vec)
  [sigma_bar_w_tilt_squ_1_5] -> cal theta_sigma_bar_w_tilt agent 5/2(sigma_bar_w_tilt_squ_1_5)
  choose ksi_est_err 18/1(y) -> cal abs 18/1(x)
  Interpreted MATLAB Function50/1 -> trans to column51/1(x)
  cal d_sigma_w agent 4/1(d_sigma_w_4) -> Integrator49/1
  Constant240/1 -> cal dw_hat agent 5/1(h3w)
  Constant195/1 -> cal theta_sigma_bar_w_tilt agent 2/1(alfa_theta_obs_w)
  Constant192/1 -> Mux67/2
  Mux71/1 -> Interpreted MATLAB Function55/1
  Constant193/1 -> cal theta_sigma_bar_w_tilt agent 1/1(alfa_theta_obs_w)
  cal differentiator d_sigma_bar_w_hat agent 4/2(Out2) -> Demux89/1, [d_sigma_bar_w_est_4], Display92/1
  Mux69/1 -> Interpreted MATLAB Function53/1
  Interpreted MATLAB Function58/1 -> trans to column59/1(x)
  [theta_sigma_bar_w_tilt_1_5] -> combine theta_sigma_bar_w_tilt/5(theta_sigma_bar_w_tilt_1_5)
  trans to column56/1(y) -> [sigma_bar_w_tilt_squ_2_4], Display106/1
  [sigma_bar_w_tilt_vec] -> choose ksi_est_err 12/1(x)
  [sigma_bar_w_tilt_vec] -> choose ksi_est_err 16/1(x)
  Constant204/1 -> Mux75/3
  choose ksi_est_err 15/1(y) -> cal abs 15/1(x)
  Constant200/1 -> cal theta_sigma_bar_w_tilt agent 3/1(alfa_theta_obs_w)
  choose ksi_est_err 13/1(y) -> cal abs 13/1(x)
  cal theta_sigma_bar_w_tilt agent 3/1(theta_sigma_bar_w_tilt_1_3) -> [theta_sigma_bar_w_tilt_1_3]
  [sigma_bar_w_tilt_squ_2_2] -> cal theta_sigma_bar_w_tilt agent 2/3(sigma_bar_w_tilt_squ_2_2)
  cal d_sigma_w agent 1/1(d_sigma_w_1) -> Integrator46/1
  [sigma_bar_w_tilt_squ_2_4] -> cal theta_sigma_bar_w_tilt agent 4/3(sigma_bar_w_tilt_squ_2_4)
  [sigma_bar_w_tilt_vec] -> cal theta_sigma_bar_w_tilt agent 3/4(sigma_bar_w_tilt_vec)
  Mux75/1 -> Interpreted MATLAB Function59/1
  Constant209/1 -> Mux70/3
  cal abs 20/1(y) -> Mux72/1
  [sigma_bar_w_tilt_squ_1_4] -> cal theta_sigma_bar_w_tilt agent 4/2(sigma_bar_w_tilt_squ_1_4)
  trans to column58/1(y) -> [sigma_bar_w_tilt_squ_2_5], Display111/1
  trans to column54/1(y) -> [sigma_bar_w_tilt_squ_2_3], Display103/1
  cal theta_sigma_bar_w_tilt agent 5/1(theta_sigma_bar_w_tilt_1_5) -> [theta_sigma_bar_w_tilt_1_5]
  trans to column51/1(y) -> [sigma_bar_w_tilt_squ_2_1], Display97/1
  cal theta_sigma_bar_w_tilt agent 1/2(theta_sigma_bar_w_tilt_2_1) -> [theta_sigma_bar_w_tilt_2_1]
  [theta_sigma_bar_w_tilt_1_4] -> combine theta_sigma_bar_w_tilt/4(theta_sigma_bar_w_tilt_1_4)
  trans to column59/1(y) -> [sigma_bar_w_tilt_squ_1_2], Display102/1
  Demux91/3 -> d_sigma_bar_w_est_5/3
  Constant242/1 -> cal d_sigma_w agent 4/1(h3w)
  [theta_sigma_bar_w_tilt_2_4] -> combine theta_sigma_bar_w_tilt/9(theta_sigma_bar_w_tilt_2_4)
  [sigma_bar_w_tilt_vec] -> choose ksi_est_err 11/1(x)
  [theta_sigma_bar_w_tilt_1_2] -> combine theta_sigma_bar_w_tilt/2(theta_sigma_bar_w_tilt_1_2)
  Constant217/1 -> Mux66/2
  combine theta_sigma_bar_w_tilt/2(theta_sigma_bar_w_tilt_2_vec) -> [theta_sigma_bar_w_tilt_2_vec]
  Interpreted MATLAB Function56/1 -> trans to column58/1(x)
  Demux86/2 -> d2_sigma_bar_w_est_3/2
  choose ksi_est_err 19/1(y) -> cal abs 19/1(x)
  [sigma_bar_w_tilt_vec] -> choose ksi_est_err 14/1(x)
  [sigma_bar_w_tilt_squ_2_1] -> cal theta_sigma_bar_w_tilt agent 1/3(sigma_bar_w_tilt_squ_2_1)
  [theta_sigma_bar_w_tilt_1_vec] -> cal sigma_bar_w_hat agent 4/3(theta_sigma_bar_w_tilt_1_vec)
  choose ksi_est_err 14/1(y) -> cal abs 14/1(x)
  Constant224/1 -> cal sigma_bar_w_hat agent 3/1(h1w)
  [sigma_bar_w_tilt_squ_2_3] -> cal theta_sigma_bar_w_tilt agent 3/3(sigma_bar_w_tilt_squ_2_3)
  Interpreted MATLAB Function53/1 -> trans to column55/1(x)
  Mux72/1 -> Interpreted MATLAB Function56/1
  cal theta_sigma_bar_w_tilt agent 5/2(theta_sigma_bar_w_tilt_2_5) -> [theta_sigma_bar_w_tilt_2_5]
  [d_sigma_bar_w_est_4] -> combine d_sigma_bar_v_est/4(d_sigma_bar_w_est_4)
  cal dw_hat agent 4/1(dw_hat_4) -> [dw_hat_4]
  Mux67/1 -> Interpreted MATLAB Function51/1
  [d_sigma_bar_w_est_1] -> combine d_sigma_bar_v_est/1(d_sigma_bar_w_est_1)
  [d_sigma_bar_w_est_2] -> combine d_sigma_bar_v_est/2(d_sigma_bar_w_est_2)
  cal differentiator d_sigma_bar_w_hat agent 5/3(Out3) -> Demux90/1, [d2_sigma_bar_w_est_5], Display95/1
  [sigma_bar_w_tilt_vec] -> cal theta_sigma_bar_w_tilt agent 2/4(sigma_bar_w_tilt_vec)
  Constant198/1 -> Mux68/3
  cal differentiator d_sigma_bar_w_hat agent 5/1(Out1) -> Display96/1, [sigma_bar_w_est_5]
  Demux91/2 -> d_sigma_bar_w_est_5/2
  Demux89/3 -> d_sigma_bar_w_est_4/3
  Constant216/1 -> Mux67/3
  [theta_sigma_bar_w_tilt_1_3] -> combine theta_sigma_bar_w_tilt/3(theta_sigma_bar_w_tilt_1_3)
  [sigma_bar_w_vec] -> cal differentiator d_sigma_bar_w_hat agent 5/1(x)
  Demux90/3 -> d2_sigma_bar_w_est_5/3
  [sigma_bar_w_tilt_vec] -> choose ksi_est_err 17/1(x)
  Demux89/2 -> d_sigma_bar_w_est_4/2
  Constant232/1 -> cal dw_hat agent 2/2(Ji)
  cal theta_sigma_bar_w_tilt agent 3/2(theta_sigma_bar_w_tilt_2_3) -> [theta_sigma_bar_w_tilt_2_3]
  [theta_sigma_bar_w_tilt_2_vec] -> cal sigma_bar_w_hat agent 2/4(theta_sigma_bar_w_tilt_2_vec)
  [dw_hat_4] -> combine dw_hat/4(dw_hat_4)
  cal differentiator d_sigma_bar_w_hat agent 4/3(Out3) -> Demux88/1, [d2_sigma_bar_w_est_4], Display93/1
  [d_sigma_bar_w_vec] -> cal dw_hat agent 4/3(d_sigma_bar_w_vec)
  Demux87/1 -> d_sigma_bar_w_est_3/1
  [taui_vec] -> cal d_sigma_w agent 3/4(taui_vec)
  Demux89/1 -> d_sigma_bar_w_est_4/1
  trans to column55/1(y) -> [sigma_bar_w_tilt_squ_1_3], Display105/1
  Demux87/2 -> d_sigma_bar_w_est_3/2
  [sigma_bar_w_hat_3] -> combine sigma_bar_w_hat/3(sigma_bar_w_hat_3)
  Interpreted MATLAB Function55/1 -> trans to column57/1(x)
  [taui_vec] -> cal d_sigma_w agent 1/4(taui_vec)
  [theta_sigma_bar_w_tilt_2_1] -> combine theta_sigma_bar_w_tilt/6(theta_sigma_bar_w_tilt_2_1)
  Constant197/1 -> Mux68/2
  cal dw_hat agent 5/1(dw_hat_5) -> [dw_hat_5]
  Constant207/1 -> Mux71/3
  choose ksi_est_err 20/1(y) -> cal abs 20/1(x)
  [sigma_bar_w_tilt_squ_2_5] -> cal theta_sigma_bar_w_tilt agent 5/3(sigma_bar_w_tilt_squ_2_5)
  cal abs 16/1(y) -> Mux75/1
  [sigma_bar_w_tilt_vec] -> cal theta_sigma_bar_w_tilt agent 1/4(sigma_bar_w_tilt_vec)
  Demux91/1 -> d_sigma_bar_w_est_5/1
  Interpreted MATLAB Function57/1 -> trans to column60/1(x)
  cal abs 19/1(y) -> Mux74/1
  Demux82/3 -> d2_sigma_bar_w_est_1/3
  [sigma_bar_w_tilt_vec] -> choose ksi_est_err 18/1(x)
  Demux90/1 -> d2_sigma_bar_w_est_5/1
  choose ksi_est_err 16/1(y) -> cal abs 16/1(x)
  Interpreted MATLAB Function59/1 -> trans to column54/1(x)
  [theta_sigma_bar_w_tilt_1_vec] -> cal sigma_bar_w_hat agent 1/3(theta_sigma_bar_w_tilt_1_vec)
  sigma_bar_w_hat Integrator 1/1 -> [sigma_bar_w_hat_1]
  Constant233/1 -> cal dw_hat agent 3/1(h3w)
  [dw_hat_1] -> combine dw_hat/1(dw_hat_1)
  [sigma_bar_w_hat_vec] -> cal dw_hat agent 5/4(sigma_bar_w_hat_vec)
  [sigma_bar_w_tilt_squ_1_2] -> cal theta_sigma_bar_w_tilt agent 2/2(sigma_bar_w_tilt_squ_1_2)
  Constant199/1 -> Mux69/2
  [sigma_bar_w_tilt_vec] -> choose ksi_est_err 13/1(x)
  [wi_vec] -> cal d_sigma_w agent 2/3(wi_vec)
  cal differentiator d_sigma_bar_w_hat agent 5/2(Out2) -> Demux91/1, [d_sigma_bar_w_est_5], Display94/1
  Integrator48/1 -> [sigma_w_3]
  [d_sigma_bar_w_est_3] -> combine d_sigma_bar_v_est/3(d_sigma_bar_w_est_3)
  Mux68/1 -> Interpreted MATLAB Function52/1
  [theta_sigma_bar_w_tilt_1_vec] -> cal sigma_bar_w_hat agent 3/3(theta_sigma_bar_w_tilt_1_vec)
  [sigma_bar_w_vec] -> cal differentiator d_sigma_bar_w_hat agent 2/1(x)
  [sigma_bar_w_hat_vec] -> cal dw_hat agent 2/4(sigma_bar_w_hat_vec)
  [d_sigma_bar_w_vec] -> cal dw_hat agent 5/3(d_sigma_bar_w_vec)
  [dw_hat_vec] -> cal error dw_tilt/2(dw_hat_vec)
  Constant196/1 -> Mux73/3
  [sigma_bar_w_vec] -> cal differentiator d_sigma_bar_w_hat agent 1/1(x)
  cal d_sigma_w agent 5/1(d_sigma_w_5) -> Integrator50/1
  [dw_vec] -> cal error dw_tilt/1(dw_vec)
  cal dw_hat agent 1/1(dw_hat_1) -> [dw_hat_1]
  cal error dw_tilt/1(dw_tilt_vec) -> [dw_tilt_vec]
  combine sigma_bar_w_hat/1(sigma_bar_w_hat_vec) -> [sigma_bar_w_hat_vec]
  Constant231/1 -> cal dw_hat agent 2/1(h3w)
  cal theta_sigma_bar_w_tilt agent 2/2(theta_sigma_bar_w_tilt_2_2) -> [theta_sigma_bar_w_tilt_2_2]
  [sigma_bar_w_tilt_squ_1_3] -> cal theta_sigma_bar_w_tilt agent 3/2(sigma_bar_w_tilt_squ_1_3)
  Constant212/1 -> cal d_sigma_w agent 2/1(h3w)
  combine dw_hat/1(dw_hat_vec) -> [dw_hat_vec]
  Constant211/1 -> cal theta_sigma_bar_w_tilt agent 5/1(alfa_theta_obs_w)
  cal differentiator d_sigma_bar_w_hat agent 1/2(Out2) -> Demux83/1, [d_sigma_bar_w_est_1], Display104/1
  choose ksi_est_err 12/1(y) -> cal abs 12/1(x)
  [sigma_w_3] -> combine sigma_w/3(sigma_w_3)
  [dw_hat_2] -> combine dw_hat/2(dw_hat_2)
  combine d_sigma_bar_v_est/1(d_sigma_bar_w_vec) -> [d_sigma_bar_w_vec]
  [sigma_bar_w_hat_2] -> combine sigma_bar_w_hat/2(sigma_bar_w_hat_2)
  Constant201/1 -> cal d_sigma_w agent 1/2(Ji)
  [d_sigma_bar_w_vec] -> cal sigma_bar_w_hat agent 4/5(d_sigma_bar_w_vec)
  Constant223/1 -> cal d_sigma_w agent 2/2(Ji)
  Mux70/1 -> Interpreted MATLAB Function54/1
  Demux88/1 -> d2_sigma_bar_w_est_4/1
  [theta_sigma_bar_w_tilt_1_vec] -> cal sigma_bar_w_hat agent 5/3(theta_sigma_bar_w_tilt_1_vec)
  [taui_vec] -> cal d_sigma_w agent 5/4(taui_vec)
  Constant229/1 -> cal sigma_bar_w_hat agent 5/2(h2w)
  choose ksi_est_err 11/1(y) -> cal abs 11/1(x)
  Demux83/1 -> d_sigma_bar_w_est_1/1
  Constant236/1 -> cal d_sigma_w agent 3/2(Ji)
  [sigma_bar_w_vec] -> cal differentiator d_sigma_bar_w_hat agent 3/1(x)
  Constant226/1 -> cal sigma_bar_w_hat agent 4/1(h1w)
  [sigma_bar_w_tilt_vec] -> choose ksi_est_err 20/1(x)
  [sigma_w_4] -> combine sigma_w/4(sigma_w_4)
  Constant205/1 -> Mux71/2
  cal differentiator d_sigma_bar_w_hat agent 2/2(Out2) -> Demux85/1, [d_sigma_bar_w_est_2], Display110/1
  [sigma_bar_w_hat_vec] -> cal combine sigma_bar_w_tilt/2(sigma_bar_w_hat_vec)
  Demux88/2 -> d2_sigma_bar_w_est_4/2
  Constant214/1 -> Mux72/2
  Constant227/1 -> cal sigma_bar_w_hat agent 4/2(h2w)
  Constant208/1 -> Mux70/2
  cal abs 14/1(y) -> Mux68/1
  Constant219/1 -> cal sigma_bar_w_hat agent 1/1(h1w)
  Constant194/1 -> Mux73/2
  [sigma_bar_w_hat_1] -> combine sigma_bar_w_hat/1(sigma_bar_w_hat_1)
  [dw_hat_3] -> combine dw_hat/3(dw_hat_3)
  trans to column57/1(y) -> [sigma_bar_w_tilt_squ_1_4], Display109/1
  Interpreted MATLAB Function54/1 -> trans to column56/1(x)
  Demux85/2 -> d_sigma_bar_w_est_2/2
  [d_sigma_bar_w_vec] -> cal sigma_bar_w_hat agent 5/5(d_sigma_bar_w_vec)
  Constant202/1 -> Mux69/3
  Constant225/1 -> cal sigma_bar_w_hat agent 3/2(h2w)
  combine theta_sigma_bar_w_tilt/1(theta_sigma_bar_w_tilt_1_vec) -> [theta_sigma_bar_w_tilt_1_vec]
  cal differentiator d_sigma_bar_w_hat agent 1/1(Out1) -> Display91/1, [sigma_bar_w_est_1]
  cal theta_sigma_bar_w_tilt agent 2/1(theta_sigma_bar_w_tilt_1_2) -> [theta_sigma_bar_w_tilt_1_2]
  [taui_vec] -> cal d_sigma_w agent 4/4(taui_vec)
  Demux82/2 -> d2_sigma_bar_w_est_1/2
  Demux86/3 -> d2_sigma_bar_w_est_3/3
  [sigma_bar_w_tilt_squ_1_1] -> cal theta_sigma_bar_w_tilt agent 1/2(sigma_bar_w_tilt_squ_1_1)
  [sigma_bar_w_hat_4] -> combine sigma_bar_w_hat/4(sigma_bar_w_hat_4)
  Constant206/1 -> cal theta_sigma_bar_w_tilt agent 4/1(alfa_theta_obs_w)
  [theta_sigma_bar_w_tilt_2_3] -> combine theta_sigma_bar_w_tilt/8(theta_sigma_bar_w_tilt_2_3)
  cal abs 17/1(y) -> Mux71/1
  cal sigma_bar_w_hat agent 2/1(d_sigma_bar_w_hat_2) -> sigma_bar_w_hat Integrator 2/1
  Demux84/2 -> d2_sigma_bar_w_est_2/2
  cal theta_sigma_bar_w_tilt agent 4/1(theta_sigma_bar_w_tilt_1_4) -> [theta_sigma_bar_w_tilt_1_4]
  cal abs 18/1(y) -> Mux70/1
  [d_sigma_bar_w_vec] -> cal dw_hat agent 1/3(d_sigma_bar_w_vec)
  Demux86/1 -> d2_sigma_bar_w_est_3/1
  cal differentiator d_sigma_bar_w_hat agent 3/1(Out1) -> Display114/1, [sigma_bar_w_est_3]
  cal abs 15/1(y) -> Mux69/1
  [theta_sigma_bar_w_tilt_2_2] -> combine theta_sigma_bar_w_tilt/7(theta_sigma_bar_w_tilt_2_2)
  cal d_sigma_w agent 2/1(d_sigma_w_2) -> Integrator47/1
  [sigma_bar_w_vec] -> cal d_sigma_w agent 1/5(sigma_w_bar_vec)
  Demux83/2 -> d_sigma_bar_w_est_1/2
  [wi_vec] -> cal sigma_w_bar/1(wi_vec)
  Constant238/1 -> cal dw_hat agent 4/1(h3w)
  sigma_bar_w_hat Integrator 4/1 -> [sigma_bar_w_hat_4]
  [sigma_bar_w_vec] -> cal d_sigma_w agent 3/5(sigma_w_bar_vec)
  cal differentiator d_sigma_bar_w_hat agent 1/3(Out3) -> Demux82/1, [d2_sigma_bar_w_est_1], Display108/1
  cal differentiator d_sigma_bar_w_hat agent 3/2(Out2) -> Demux87/1, [d_sigma_bar_w_est_3], Display115/1
  [sigma_w_vec] -> cal sigma_w_bar/2(sigma_w_vec)
  Demux85/1 -> d_sigma_bar_w_est_2/1
  cal sigma_w_bar/1(sigma_bar_w_vec) -> [sigma_bar_w_vec]
  Constant230/1 -> cal dw_hat agent 1/1(h3w)
  Demux84/3 -> d2_sigma_bar_w_est_2/3
  Constant244/1 -> cal d_sigma_w agent 5/1(h3w)
  [sigma_bar_w_vec] -> cal d_sigma_w agent 5/5(sigma_w_bar_vec)
  cal theta_sigma_bar_w_tilt agent 4/2(theta_sigma_bar_w_tilt_2_4) -> [theta_sigma_bar_w_tilt_2_4]
  cal differentiator d_sigma_bar_w_hat agent 4/1(Out1) -> Display117/1, [sigma_bar_w_est_4]
  trans to column53/1(y) -> [sigma_bar_w_tilt_squ_2_2], Display99/1
  Integrator49/1 -> [sigma_w_4]
  Demux82/1 -> d2_sigma_bar_w_est_1/1
  cal differentiator d_sigma_bar_w_hat agent 2/1(Out1) -> Display107/1, [sigma_bar_w_est_2]
  Integrator47/1 -> [sigma_w_2]
  [sigma_w_5] -> combine sigma_w/5(sigma_w_5)
  cal combine sigma_bar_w_tilt/1(sigma_bar_w_tilt_vec) -> [sigma_bar_w_tilt_vec]
  [sigma_w_2] -> combine sigma_w/2(sigma_w_2)
  [sigma_w_1] -> combine sigma_w/1(sigma_w_1)
  Mux74/1 -> Interpreted MATLAB Function57/1
  Constant234/1 -> cal d_sigma_w agent 3/1(h3w)
  Demux87/3 -> d_sigma_bar_w_est_3/3
  Constant210/1 -> Mux74/2
  Demux84/1 -> d2_sigma_bar_w_est_2/1
  [theta_sigma_bar_w_tilt_2_vec] -> cal sigma_bar_w_hat agent 4/4(theta_sigma_bar_w_tilt_2_vec)
  [wi_vec] -> cal d_sigma_w agent 5/3(wi_vec)
  [sigma_bar_w_vec] -> cal d_sigma_w agent 4/5(sigma_w_bar_vec)
  [wi_vec] -> cal d_sigma_w agent 3/3(wi_vec)
  Mux73/1 -> Interpreted MATLAB Function58/1
  [taui_vec] -> cal d_sigma_w agent 2/4(taui_vec)
  [theta_sigma_bar_w_tilt_2_5] -> combine theta_sigma_bar_w_tilt/10(theta_sigma_bar_w_tilt_2_5)
  cal differentiator d_sigma_bar_w_hat agent 3/3(Out3) -> Demux86/1, [d2_sigma_bar_w_est_3], Display116/1
  Integrator50/1 -> [sigma_w_5]
  Constant239/1 -> cal dw_hat agent 4/2(Ji)
  cal differentiator d_sigma_bar_w_hat agent 2/3(Out3) -> Demux84/1, [d2_sigma_bar_w_est_2], Display113/1
  [theta_sigma_bar_w_tilt_1_1] -> combine theta_sigma_bar_w_tilt/1(theta_sigma_bar_w_tilt_1_1)
  Constant243/1 -> cal d_sigma_w agent 4/2(Ji)
  Demux83/3 -> d_sigma_bar_w_est_1/3
  [sigma_bar_w_vec] -> cal d_sigma_w agent 2/5(sigma_w_bar_vec)
  [sigma_bar_w_tilt_vec] -> cal theta_sigma_bar_w_tilt agent 4/4(sigma_bar_w_tilt_vec)
  cal sigma_bar_w_hat agent 4/1(d_sigma_bar_w_hat_4) -> sigma_bar_w_hat Integrator 4/1
  Constant191/1 -> cal d_sigma_w agent 5/2(Ji)
  Mux66/1 -> Interpreted MATLAB Function50/1
  cal taui agent 1/1(tau_1) -> [tau_1]
  [dw_vec] -> wi dynam agent 1/4(dw_vec)
  [dw_vec] -> wi dynam agent 2/4(dw_vec)
  [dw_vec] -> wi dynam agent 3/4(dw_vec)
  [dw_vec] -> wi dynam agent 4/4(dw_vec)
  [dw_vec] -> wi dynam agent 5/4(dw_vec)
  [sgi_vec] -> E_sgi agent 1/1(sgi_vec)
  E_sgi agent 1/1(E_sgi_1) -> [E_sgi_1]
  combine E_sgi_vec/1(E_sgi_vec) -> Memory9/1
  [E_sgi_1] -> combine E_sgi_vec/1(E_sgi_1)
  [E_sgi_2] -> combine E_sgi_vec/2(E_sgi_2)
  [E_sgi_3] -> combine E_sgi_vec/3(E_sgi_3)
  [E_sgi_4] -> combine E_sgi_vec/4(E_sgi_4)
  [E_sgi_5] -> combine E_sgi_vec/5(E_sgi_5)
  Memory9/1 -> [E_sgi_vec]
  [sgi_vec] -> E_sgi agent 2/1(sgi_vec)
  sgi dynam agent 2/1(dsgi_2) -> Integrator16/1
  Integrator16/1 -> [sgi_2]
  cal Ri agent 2/1(Ri_2) -> [Ri_2]
  [wi_vec] -> sgi dynam agent 2/2(wi_vec)
  [E_sgi_vec] -> sgi dynam agent 2/1(E_sgi_vec)
  E_sgi agent 2/1(E_sgi_2) -> [E_sgi_2]
  [sgi_vec] -> cal Ri agent 2/1(sgi_vec)
  Integrator18/1 -> [sgi_3]
  [E_sgi_vec] -> sgi dynam agent 3/1(E_sgi_vec)
  cal Ri agent 3/1(Ri_3) -> [Ri_3]
  E_sgi agent 3/1(E_sgi_3) -> [E_sgi_3]
  sgi dynam agent 3/1(dsgi_3) -> Integrator18/1
  [sgi_vec] -> cal Ri agent 3/1(sgi_vec)
  [sgi_vec] -> E_sgi agent 3/1(sgi_vec)
  [wi_vec] -> sgi dynam agent 3/2(wi_vec)
  [sgi_vec] -> cal Ri agent 4/1(sgi_vec)
  sgi dynam agent 4/1(dsgi_4) -> Integrator27/1
  E_sgi agent 4/1(E_sgi_4) -> [E_sgi_4]
  [E_sgi_vec] -> sgi dynam agent 4/1(E_sgi_vec)
  Integrator27/1 -> [sgi_4]
  [wi_vec] -> sgi dynam agent 4/2(wi_vec)
  [sgi_vec] -> E_sgi agent 4/1(sgi_vec)
  cal Ri agent 4/1(Ri_4) -> [Ri_4]
  [E_sgi_vec] -> sgi dynam agent 5/1(E_sgi_vec)
  sgi dynam agent 5/1(dsgi_5) -> Integrator28/1
  E_sgi agent 5/1(E_sgi_5) -> [E_sgi_5]
  [sgi_vec] -> cal Ri agent 5/1(sgi_vec)
  [wi_vec] -> sgi dynam agent 5/2(wi_vec)
  Integrator28/1 -> [sgi_5]
  cal Ri agent 5/1(Ri_5) -> [Ri_5]
  [sgi_vec] -> E_sgi agent 5/1(sgi_vec)
  [sgei_vec] -> E_sgei agent 1/1(sgei_vec)
  E_sgei agent 1/1(E_sgei_1) -> [E_sgei_1]
  [sgei_vec] -> cal Rei agent 1/1(sgei_vec)
  cal Rei agent 1/1(Rei_1) -> [Rei_1]
  cal Rei agent 2/1(Rei_2) -> [Rei_2]
  [Rei_vec] -> cal wei agent 2/2(Rei_vec)
  cal wei agent 2/1(wei_2) -> [wei_2]
  E_sgei agent 2/1(E_sgei_2) -> [E_sgei_2]
  [wci_vec] -> cal wei agent 2/3(wci_vec)
  [E_sgei_vec] -> dsgei dynam agent 2/1(E_sgei_vec)
  [wi_vec] -> cal wei agent 2/1(wi_vec)
  Integrator29/1 -> [sgei_2]
  dsgei dynam agent 2/1(dsgei_2) -> Integrator29/1
  [sgei_vec] -> E_sgei agent 2/1(sgei_vec)
  [sgei_vec] -> cal Rei agent 2/1(sgei_vec)
  [wei_vec] -> dsgei dynam agent 2/2(wei_vec)
  [wci_vec] -> cal wei agent 3/3(wci_vec)
  [wei_vec] -> dsgei dynam agent 3/2(wei_vec)
  [sgei_vec] -> cal Rei agent 3/1(sgei_vec)
  dsgei dynam agent 3/1(dsgei_3) -> Integrator30/1
  [wi_vec] -> cal wei agent 3/1(wi_vec)
  [E_sgei_vec] -> dsgei dynam agent 3/1(E_sgei_vec)
  [sgei_vec] -> E_sgei agent 3/1(sgei_vec)
  cal Rei agent 3/1(Rei_3) -> [Rei_3]
  cal wei agent 3/1(wei_3) -> [wei_3]
  [Rei_vec] -> cal wei agent 3/2(Rei_vec)
  Integrator30/1 -> [sgei_3]
  E_sgei agent 3/1(E_sgei_3) -> [E_sgei_3]
  [wei_vec] -> dsgei dynam agent 4/2(wei_vec)
  [wci_vec] -> cal wei agent 4/3(wci_vec)
  [sgei_vec] -> cal Rei agent 4/1(sgei_vec)
  [wi_vec] -> cal wei agent 4/1(wi_vec)
  [Rei_vec] -> cal wei agent 4/2(Rei_vec)
  [sgei_vec] -> E_sgei agent 4/1(sgei_vec)
  dsgei dynam agent 4/1(dsgei_4) -> Integrator32/1
  cal Rei agent 4/1(Rei_4) -> [Rei_4]
  cal wei agent 4/1(wei_4) -> [wei_4]
  Integrator32/1 -> [sgei_4]
  E_sgei agent 4/1(E_sgei_4) -> [E_sgei_4]
  [E_sgei_vec] -> dsgei dynam agent 4/1(E_sgei_vec)
  [E_sgei_vec] -> dsgei dynam agent 5/1(E_sgei_vec)
  E_sgei agent 5/1(E_sgei_5) -> [E_sgei_5]
  cal Rei agent 5/1(Rei_5) -> [Rei_5]
  [sgei_vec] -> E_sgei agent 5/1(sgei_vec)
  [Rei_vec] -> cal wei agent 5/2(Rei_vec)
  cal wei agent 5/1(wei_5) -> [wei_5]
  dsgei dynam agent 5/1(dsgei_5) -> Integrator33/1
  [wci_vec] -> cal wei agent 5/3(wci_vec)
  [sgei_vec] -> cal Rei agent 5/1(sgei_vec)
  [wei_vec] -> dsgei dynam agent 5/2(wei_vec)
  [wi_vec] -> cal wei agent 5/1(wi_vec)
  Integrator33/1 -> [sgei_5]
  [E_sgei_1] -> combine E_sgi_vec1/1(E_sgei_1)
  Memory10/1 -> [E_sgei_vec]
  [E_sgei_4] -> combine E_sgi_vec1/4(E_sgei_4)
  combine E_sgi_vec1/1(E_sgei_vec) -> Memory10/1
  [E_sgei_2] -> combine E_sgi_vec1/2(E_sgei_2)
  [E_sgei_5] -> combine E_sgi_vec1/5(E_sgei_5)
  [E_sgei_3] -> combine E_sgi_vec1/3(E_sgei_3)
  [wi_vec] -> cal Gamma_wi agent 1/1(wi_vec)
  cal Gamma_wi agent 1/1(Gamma_wi_1) -> [Gamma_wi_1]
  cal Gamma_wi agent 2/1(Gamma_wi_2) -> [Gamma_wi_2]
  [wi_vec] -> cal Gamma_wi agent 2/1(wi_vec)
  [wi_vec] -> cal Gamma_wi agent 3/1(wi_vec)
  cal Gamma_wi agent 3/1(Gamma_wi_3) -> [Gamma_wi_3]
  cal Gamma_wi agent 4/1(Gamma_wi_4) -> [Gamma_wi_4]
  [wi_vec] -> cal Gamma_wi agent 4/1(wi_vec)
  [wi_vec] -> cal Gamma_wi agent 5/1(wi_vec)
  cal Gamma_wi agent 5/1(Gamma_wi_5) -> [Gamma_wi_5]
  [Gamma_wi_4] -> combine Gamma_wi_vec/4(Gamma_wi_4)
  combine Gamma_wi_vec/1(Gamma_wi_vec) -> Memory11/1
  [Gamma_wi_2] -> combine Gamma_wi_vec/2(Gamma_wi_2)
  [Gamma_wi_1] -> combine Gamma_wi_vec/1(Gamma_wi_1)
  [Gamma_wi_3] -> combine Gamma_wi_vec/3(Gamma_wi_3)
  [Gamma_wi_5] -> combine Gamma_wi_vec/5(Gamma_wi_5)
  Memory11/1 -> [Gamma_wi_vec]
  [wei_vec] -> cal Fi agent 1/1(wei_vec)
  [Rei_vec] -> cal Fi agent 1/2(Rei_vec)
  [wci_vec] -> cal Fi agent 1/3(wci_vec)
  [dwci_vec] -> cal Fi agent 1/4(dwci_vec)
  cal Fi agent 1/1(Fi_1) -> [Fi_1]
  [Rei_vec] -> cal Fi agent 2/2(Rei_vec)
  [wci_vec] -> cal Fi agent 2/3(wci_vec)
  [wei_vec] -> cal Fi agent 2/1(wei_vec)
  cal Fi agent 2/1(Fi_2) -> [Fi_2]
  [dwci_vec] -> cal Fi agent 2/4(dwci_vec)
  [dwci_vec] -> cal Fi agent 3/4(dwci_vec)
  cal Fi agent 3/1(Fi_3) -> [Fi_3]
  [wci_vec] -> cal Fi agent 3/3(wci_vec)
  [Rei_vec] -> cal Fi agent 3/2(Rei_vec)
  [wei_vec] -> cal Fi agent 3/1(wei_vec)
  [dwci_vec] -> cal Fi agent 4/4(dwci_vec)
  [wei_vec] -> cal Fi agent 4/1(wei_vec)
  [Rei_vec] -> cal Fi agent 4/2(Rei_vec)
  [wci_vec] -> cal Fi agent 4/3(wci_vec)
  cal Fi agent 4/1(Fi_4) -> [Fi_4]
  [wei_vec] -> cal Fi agent 5/1(wei_vec)
  [wci_vec] -> cal Fi agent 5/3(wci_vec)
  [dwci_vec] -> cal Fi agent 5/4(dwci_vec)
  cal Fi agent 5/1(Fi_5) -> [Fi_5]
  [Rei_vec] -> cal Fi agent 5/2(Rei_vec)
  [Fi_1] -> combine Fi_vec/1(Fi_1)
  [Fi_4] -> combine Fi_vec/4(Fi_4)
  combine Fi_vec/1(Fi_vec) -> Memory13/1
  [Fi_3] -> combine Fi_vec/3(Fi_3)
  Memory13/1 -> [Fi_vec]
  [Fi_2] -> combine Fi_vec/2(Fi_2)
  [Fi_5] -> combine Fi_vec/5(Fi_5)
  Memory16/1 -> [Gamma_Fi_vec]
  cal Gamma_Fi agent 1/1(Gamma_Fi_1) -> [Gamma_Fi_1]
  [Fi_vec] -> cal Gamma_Fi agent 1/1(Fi_vec)
  [Gamma_Fi_1] -> combine Gamma_Fi_vec/1(Gamma_Fi_1)
  [Gamma_Fi_4] -> combine Gamma_Fi_vec/4(Gamma_Fi_4)
  combine Gamma_Fi_vec/1(Gamma_Fi_vec) -> Memory16/1
  [Gamma_Fi_3] -> combine Gamma_Fi_vec/3(Gamma_Fi_3)
  [Gamma_Fi_2] -> combine Gamma_Fi_vec/2(Gamma_Fi_2)
  [Gamma_Fi_5] -> combine Gamma_Fi_vec/5(Gamma_Fi_5)
  cal Gamma_Fi agent 2/1(Gamma_Fi_2) -> [Gamma_Fi_2]
  [Fi_vec] -> cal Gamma_Fi agent 2/1(Fi_vec)
  [Fi_vec] -> cal Gamma_Fi agent 3/1(Fi_vec)
  cal Gamma_Fi agent 3/1(Gamma_Fi_3) -> [Gamma_Fi_3]
  [Fi_vec] -> cal Gamma_Fi agent 4/1(Fi_vec)
  cal Gamma_Fi agent 4/1(Gamma_Fi_4) -> [Gamma_Fi_4]
  cal Gamma_Fi agent 5/1(Gamma_Fi_5) -> [Gamma_Fi_5]
  [Fi_vec] -> cal Gamma_Fi agent 5/1(Fi_vec)
  Constant1/1 -> cal zetai agent 1/1(l1)
  Constant2/1 -> cal zetai agent 1/2(l2)
  Constant3/1 -> cal zetai agent 1/3(ksg)
  [zetai_vec] -> cal zetai agent 1/4(zetai_vec)
  [sgei_vec] -> cal zetai agent 1/5(sgei_vec)
  cal zetai agent 1/1(d_zetai_1) -> [d_zetai_1], Integrator34/1
  Integrator34/1 -> [zetai_1]
  Constant4/1 -> cal zetai agent 2/1(l1)
  Integrator35/1 -> [zetai_2]
  Constant5/1 -> cal zetai agent 2/2(l2)
  Constant6/1 -> cal zetai agent 2/3(ksg)
  cal zetai agent 2/1(d_zetai_2) -> [d_zetai_2], Integrator35/1
  [zetai_vec] -> cal zetai agent 2/4(zetai_vec)
  [sgei_vec] -> cal zetai agent 2/5(sgei_vec)
  Integrator36/1 -> [zetai_3]
  [zetai_vec] -> cal zetai agent 3/4(zetai_vec)
  Constant9/1 -> cal zetai agent 3/3(ksg)
  Constant8/1 -> cal zetai agent 3/2(l2)
  cal zetai agent 3/1(d_zetai_3) -> [d_zetai_3], Integrator36/1
  [sgei_vec] -> cal zetai agent 3/5(sgei_vec)
  Constant7/1 -> cal zetai agent 3/1(l1)
  [sgei_vec] -> cal zetai agent 4/5(sgei_vec)
  Integrator37/1 -> [zetai_4]
  Constant10/1 -> cal zetai agent 4/1(l1)
  Constant11/1 -> cal zetai agent 4/2(l2)
  Constant12/1 -> cal zetai agent 4/3(ksg)
  [zetai_vec] -> cal zetai agent 4/4(zetai_vec)
  cal zetai agent 4/1(d_zetai_4) -> [d_zetai_4], Integrator37/1
  [zetai_vec] -> cal zetai agent 5/4(zetai_vec)
  Constant15/1 -> cal zetai agent 5/3(ksg)
  Constant14/1 -> cal zetai agent 5/2(l2)
  Constant13/1 -> cal zetai agent 5/1(l1)
  Integrator38/1 -> [zetai_5]
  [sgei_vec] -> cal zetai agent 5/5(sgei_vec)
  cal zetai agent 5/1(d_zetai_5) -> [d_zetai_5], Integrator38/1
  [zetai_2] -> combine zetai_vec/2(zetai_2)
  [zetai_3] -> combine zetai_vec/3(zetai_3)
  Memory17/1 -> [zetai_vec]
  combine zetai_vec/1(zetai_vec) -> Memory17/1
  [zetai_5] -> combine zetai_vec/5(zetai_5)
  [zetai_1] -> combine zetai_vec/1(zetai_1)
  [zetai_4] -> combine zetai_vec/4(zetai_4)
  [d_zetai_4] -> combine d_zetai_vec/4(d_zetai_4)
  [d_zetai_5] -> combine d_zetai_vec/5(d_zetai_5)
  Memory18/1 -> [d_zetai_vec]
  [d_zetai_1] -> combine d_zetai_vec/1(d_zetai_1)
  combine d_zetai_vec/1(d_zetai_vec) -> Memory18/1
  [d_zetai_2] -> combine d_zetai_vec/2(d_zetai_2)
  [d_zetai_3] -> combine d_zetai_vec/3(d_zetai_3)
  [Gamma_Fi_vec] -> cal Gamma_Fi_min_dzetai agent 1/1(Gamma_Fi_vec)
  [d_zetai_vec] -> cal Gamma_Fi_min_dzetai agent 1/2(d_zetai_vec)
  cal Gamma_Fi_min_dzetai agent 1/1(Gamma_Fi_min_dzetai_1) -> [Gamma_Fi_min_dzetai_1]
  [d_zetai_vec] -> cal Gamma_Fi_min_dzetai agent 2/2(d_zetai_vec)
  [Gamma_Fi_vec] -> cal Gamma_Fi_min_dzetai agent 2/1(Gamma_Fi_vec)
  cal Gamma_Fi_min_dzetai agent 2/1(Gamma_Fi_min_dzetai_2) -> [Gamma_Fi_min_dzetai_2]
  cal Gamma_Fi_min_dzetai agent 3/1(Gamma_Fi_min_dzetai_3) -> [Gamma_Fi_min_dzetai_3]
  [d_zetai_vec] -> cal Gamma_Fi_min_dzetai agent 3/2(d_zetai_vec)
  [Gamma_Fi_vec] -> cal Gamma_Fi_min_dzetai agent 3/1(Gamma_Fi_vec)
  [Gamma_Fi_vec] -> cal Gamma_Fi_min_dzetai agent 4/1(Gamma_Fi_vec)
  cal Gamma_Fi_min_dzetai agent 4/1(Gamma_Fi_min_dzetai_4) -> [Gamma_Fi_min_dzetai_4]
  [d_zetai_vec] -> cal Gamma_Fi_min_dzetai agent 4/2(d_zetai_vec)
  [d_zetai_vec] -> cal Gamma_Fi_min_dzetai agent 5/2(d_zetai_vec)
  [Gamma_Fi_vec] -> cal Gamma_Fi_min_dzetai agent 5/1(Gamma_Fi_vec)
  cal Gamma_Fi_min_dzetai agent 5/1(Gamma_Fi_min_dzetai_5) -> [Gamma_Fi_min_dzetai_5]
  [Gamma_Fi_min_dzetai_2] -> combine Gamma_Fi_min_dzetai/2(Gamma_Fi_min_dzetai_2)
  [Gamma_Fi_min_dzetai_3] -> combine Gamma_Fi_min_dzetai/3(Gamma_Fi_min_dzetai_3)
  Memory19/1 -> [Gamma_Fi_min_dzetai_vec]
  combine Gamma_Fi_min_dzetai/1(Gamma_Fi_min_dzetai_vec) -> Memory19/1
  [Gamma_Fi_min_dzetai_5] -> combine Gamma_Fi_min_dzetai/5(Gamma_Fi_min_dzetai_5)
  [Gamma_Fi_min_dzetai_1] -> combine Gamma_Fi_min_dzetai/1(Gamma_Fi_min_dzetai_1)
  [Gamma_Fi_min_dzetai_4] -> combine Gamma_Fi_min_dzetai/4(Gamma_Fi_min_dzetai_4)
  [wi_vec] -> cal thetai_hat agent 1/2(wi_vec)
  Constant16/1 -> cal thetai_hat agent 1/1(mu)
  [wei_vec] -> cal thetai_hat agent 1/3(wei_vec)
  [zetai_vec] -> cal thetai_hat agent 1/4(zetai_vec)
  [Gamma_Fi_min_dzetai_vec] -> cal thetai_hat agent 1/5(Gamma_Fi_min_dzetai_vec)
  [Gamma_wi_vec] -> cal thetai_hat agent 1/6(Gamma_wi_vec)
  cal thetai_hat agent 1/1(d_thetai_hat_1) -> Integrator39/1
  Integrator39/1 -> [thetai_hat_1]
  Integrator40/1 -> [thetai_hat_2]
  [zetai_vec] -> cal thetai_hat agent 2/4(zetai_vec)
  cal thetai_hat agent 2/1(d_thetai_hat_2) -> Integrator40/1
  [wei_vec] -> cal thetai_hat agent 2/3(wei_vec)
  [Gamma_Fi_min_dzetai_vec] -> cal thetai_hat agent 2/5(Gamma_Fi_min_dzetai_vec)
  [Gamma_wi_vec] -> cal thetai_hat agent 2/6(Gamma_wi_vec)
  [wi_vec] -> cal thetai_hat agent 2/2(wi_vec)
  Constant17/1 -> cal thetai_hat agent 2/1(mu)
  [wei_vec] -> cal thetai_hat agent 3/3(wei_vec)
  [wi_vec] -> cal thetai_hat agent 3/2(wi_vec)
  Constant18/1 -> cal thetai_hat agent 3/1(mu)
  cal thetai_hat agent 3/1(d_thetai_hat_3) -> Integrator41/1
  [Gamma_Fi_min_dzetai_vec] -> cal thetai_hat agent 3/5(Gamma_Fi_min_dzetai_vec)
  [zetai_vec] -> cal thetai_hat agent 3/4(zetai_vec)
  Integrator41/1 -> [thetai_hat_3]
  [Gamma_wi_vec] -> cal thetai_hat agent 3/6(Gamma_wi_vec)
  [zetai_vec] -> cal thetai_hat agent 4/4(zetai_vec)
  [Gamma_Fi_min_dzetai_vec] -> cal thetai_hat agent 4/5(Gamma_Fi_min_dzetai_vec)
  [wi_vec] -> cal thetai_hat agent 4/2(wi_vec)
  [wei_vec] -> cal thetai_hat agent 4/3(wei_vec)
  [Gamma_wi_vec] -> cal thetai_hat agent 4/6(Gamma_wi_vec)
  cal thetai_hat agent 4/1(d_thetai_hat_4) -> Integrator43/1
  Constant19/1 -> cal thetai_hat agent 4/1(mu)
  Integrator43/1 -> [thetai_hat_4]
  Integrator45/1 -> [thetai_hat_5]
  cal thetai_hat agent 5/1(d_thetai_hat_5) -> Integrator45/1
  [wi_vec] -> cal thetai_hat agent 5/2(wi_vec)
  [zetai_vec] -> cal thetai_hat agent 5/4(zetai_vec)
  [Gamma_Fi_min_dzetai_vec] -> cal thetai_hat agent 5/5(Gamma_Fi_min_dzetai_vec)
  [Gamma_wi_vec] -> cal thetai_hat agent 5/6(Gamma_wi_vec)
  [wei_vec] -> cal thetai_hat agent 5/3(wei_vec)
  Constant20/1 -> cal thetai_hat agent 5/1(mu)
  [thetai_hat_2] -> combine thetai_hat/2(thetai_hat_2)
  combine thetai_hat/1(thetai_hat_vec) -> Memory20/1
  [thetai_hat_4] -> combine thetai_hat/4(thetai_hat_4)
  [thetai_hat_1] -> combine thetai_hat/1(thetai_hat_1)
  [thetai_hat_5] -> combine thetai_hat/5(thetai_hat_5)
  Memory20/1 -> [thetai_hat_vec]
  [thetai_hat_3] -> combine thetai_hat/3(thetai_hat_3)
  Constant21/1 -> cal taui agent 1/1(kw)
  Constant22/1 -> cal taui agent 1/2(ksg)
  [wi_vec] -> cal taui agent 1/3(wi_vec)
  [wei_vec] -> cal taui agent 1/4(wei_vec)
  [zetai_vec] -> cal taui agent 1/5(zetai_vec)
  [sgei_vec] -> cal taui agent 1/6(sgei_vec)
  [dw_hat_vec] -> cal taui agent 1/7(dw_hat_vec)
  [thetai_hat_vec] -> cal taui agent 1/8(thetai_hat_vec)
  [Gamma_wi_vec] -> cal taui agent 1/9(Gamma_wi_vec)
  [Gamma_Fi_min_dzetai_vec] -> cal taui agent 1/10(Gamma_Fi_min_dzetai_vec)
  [thetai_hat_vec] -> cal taui agent 2/8(thetai_hat_vec)
  [Gamma_wi_vec] -> cal taui agent 2/9(Gamma_wi_vec)
  [wi_vec] -> cal taui agent 2/3(wi_vec)
  [sgei_vec] -> cal taui agent 2/6(sgei_vec)
  [wei_vec] -> cal taui agent 2/4(wei_vec)
  [zetai_vec] -> cal taui agent 2/5(zetai_vec)
  Constant24/1 -> cal taui agent 2/2(ksg)
  Constant23/1 -> cal taui agent 2/1(kw)
  [dw_hat_vec] -> cal taui agent 2/7(dw_hat_vec)
  [Gamma_Fi_min_dzetai_vec] -> cal taui agent 2/10(Gamma_Fi_min_dzetai_vec)
  cal taui agent 2/1(tau_2) -> [tau_2]
  [dw_hat_vec] -> cal taui agent 3/7(dw_hat_vec)
  Constant25/1 -> cal taui agent 3/1(kw)
  [zetai_vec] -> cal taui agent 3/5(zetai_vec)
  [sgei_vec] -> cal taui agent 3/6(sgei_vec)
  [Gamma_Fi_min_dzetai_vec] -> cal taui agent 3/10(Gamma_Fi_min_dzetai_vec)
  [Gamma_wi_vec] -> cal taui agent 3/9(Gamma_wi_vec)
  [wei_vec] -> cal taui agent 3/4(wei_vec)
  [wi_vec] -> cal taui agent 3/3(wi_vec)
  [thetai_hat_vec] -> cal taui agent 3/8(thetai_hat_vec)
  Constant26/1 -> cal taui agent 3/2(ksg)
  cal taui agent 3/1(tau_3) -> [tau_3]
  [wi_vec] -> cal taui agent 4/3(wi_vec)
  [Gamma_wi_vec] -> cal taui agent 4/9(Gamma_wi_vec)
  [wei_vec] -> cal taui agent 4/4(wei_vec)
  [sgei_vec] -> cal taui agent 4/6(sgei_vec)
  Constant28/1 -> cal taui agent 4/2(ksg)
  Constant27/1 -> cal taui agent 4/1(kw)
  [dw_hat_vec] -> cal taui agent 4/7(dw_hat_vec)
  [zetai_vec] -> cal taui agent 4/5(zetai_vec)
  [thetai_hat_vec] -> cal taui agent 4/8(thetai_hat_vec)
  [Gamma_Fi_min_dzetai_vec] -> cal taui agent 4/10(Gamma_Fi_min_dzetai_vec)
  cal taui agent 4/1(tau_4) -> [tau_4]
  [dw_hat_vec] -> cal taui agent 5/7(dw_hat_vec)
  [thetai_hat_vec] -> cal taui agent 5/8(thetai_hat_vec)
  Constant29/1 -> cal taui agent 5/1(kw)
  Constant30/1 -> cal taui agent 5/2(ksg)
  [sgei_vec] -> cal taui agent 5/6(sgei_vec)
  [wei_vec] -> cal taui agent 5/4(wei_vec)
  [zetai_vec] -> cal taui agent 5/5(zetai_vec)
  [Gamma_wi_vec] -> cal taui agent 5/9(Gamma_wi_vec)
  [wi_vec] -> cal taui agent 5/3(wi_vec)
  [Gamma_Fi_min_dzetai_vec] -> cal taui agent 5/10(Gamma_Fi_min_dzetai_vec)
  cal taui agent 5/1(tau_5) -> [tau_5]
  [Ri_vec] -> cal Rci agent 1/1(Ri_vec)
  [Rei_vec] -> cal Rci agent 1/2(Rei_vec)
  cal Rci agent 1/1(Rci_1) -> [Rci_1]
  cal Rci agent 2/1(Rci_2) -> [Rci_2]
  [Rei_vec] -> cal Rci agent 2/2(Rei_vec)
  [Ri_vec] -> cal Rci agent 2/1(Ri_vec)
  [Ri_vec] -> cal Rci agent 3/1(Ri_vec)
  cal Rci agent 3/1(Rci_3) -> [Rci_3]
  [Rei_vec] -> cal Rci agent 3/2(Rei_vec)
  [Ri_vec] -> cal Rci agent 4/1(Ri_vec)
  [Rei_vec] -> cal Rci agent 4/2(Rei_vec)
  cal Rci agent 4/1(Rci_4) -> [Rci_4]
  cal Rci agent 5/1(Rci_5) -> [Rci_5]
  [Rei_vec] -> cal Rci agent 5/2(Rei_vec)
  [Ri_vec] -> cal Rci agent 5/1(Ri_vec)
  [Rci_3] -> combine Rci/3(Rci_3)
  combine Rci/1(Rci_vec) -> Memory21/1
  [Rci_4] -> combine Rci/4(Rci_4)
  [Rci_2] -> combine Rci/2(Rci_2)
  [Rci_1] -> combine Rci/1(Rci_1)
  Memory21/1 -> [Rci_vec]
  [Rci_5] -> combine Rci/5(Rci_5)
  [zetai_vec] -> depart zetai_3/1(x), depart zetai_5/1(x), depart zetai_4/1(x), depart zetai_2/1(x), depart zetai_1/1(x)
  depart zetai_3/1(y) -> Display8/1, Demux30/1
  depart zetai_2/1(y) -> Display7/1, Demux29/1
  depart zetai_1/1(y) -> Display6/1, Demux28/1
  depart zetai_5/1(y) -> Display10/1, Demux32/1
  depart zetai_4/1(y) -> Display9/1, Demux31/1
  depart theta_hat_2/1(y) -> Demux58/1, Display13/1
  [thetai_hat_vec] -> depart theta_hat_3/1(x), depart theta_hat_5/1(x), depart theta_hat_4/1(x), depart theta_hat_2/1(x), depart theta_hat_1/1(x)
  depart theta_hat_1/1(y) -> Display12/1, Demux57/1
  [wei_node_1] -> Demux67/1
  Mux/1 -> Scope7/1
  Mux1/1 -> Scope7/2
  Mux2/1 -> Scope7/3
  Demux28/1 -> Mux/1
  Demux28/2 -> Mux1/1
  Demux28/3 -> Mux2/1
  Demux67/1 -> Mux/2
  Demux67/2 -> Mux1/2
  Demux67/3 -> Mux2/2
  Mux4/1 -> Scope8/2
  Mux3/1 -> Scope8/1
  Mux5/1 -> Scope8/3
  Demux68/1 -> Mux3/2
  Demux68/2 -> Mux4/2
  Demux68/3 -> Mux5/2
  Demux29/1 -> Mux3/1
  Demux29/2 -> Mux4/1
  Demux29/3 -> Mux5/1
  [wei_node_2] -> Demux68/1
  Mux36/1 -> Scope9/1
  Mux37/1 -> Scope9/2
  Mux38/1 -> Scope9/3
  Demux30/1 -> Mux36/1
  Demux30/2 -> Mux37/1
  Demux30/3 -> Mux38/1
  Demux69/1 -> Mux36/2
  Demux69/3 -> Mux38/2
  Demux69/2 -> Mux37/2
  [wei_node_3] -> Demux69/1
  Mux39/1 -> Scope10/1
  Mux40/1 -> Scope10/2
  Mux56/1 -> Scope10/3
  Demux70/2 -> Mux40/2
  Demux70/1 -> Mux39/2
  Demux70/3 -> Mux56/2
  [wei_node_4] -> Demux70/1
  Demux31/1 -> Mux39/1
  Demux31/2 -> Mux40/1
  Demux31/3 -> Mux56/1
  Mux57/1 -> Scope11/1
  Mux58/1 -> Scope11/2
  Mux59/1 -> Scope11/3
  Demux71/1 -> Mux57/2
  Demux71/2 -> Mux58/2
  Demux71/3 -> Mux59/2
  [wei_node_5] -> Demux71/1
  Demux32/1 -> Mux57/1
  Demux32/2 -> Mux58/1
  Demux32/3 -> Mux59/1
  depart Ji_1_1/1(y) -> [Ji_1_1]
  depart Ji_2_2/1(y) -> [Ji_2_2]
  depart Ji_3_3/1(y) -> [Ji_3_3]
  depart Ji_2_3/1(y) -> [Ji_2_3]
  Constant31/1 -> depart Ji_1_2/1(x), depart Ji_1_3/1(x), depart Ji_2_3/1(x), depart Ji_3_3/1(x), depart Ji_2_2/1(x), depart Ji_1_1/1(x)
  depart Ji_1_3/1(y) -> [Ji_1_3]
  depart Ji_1_2/1(y) -> [Ji_1_2]
  Mux65/1 -> Scope30/3
  Mux64/1 -> Scope30/2
  Mux63/1 -> Scope30/1
  Mux62/1 -> Scope22/3
  Mux61/1 -> Scope22/2
  Mux60/1 -> Scope22/1
  Demux57/1 -> Mux60/1
  Demux57/2 -> Mux61/1
  Demux57/3 -> Mux62/1
  Demux57/4 -> Mux63/1
  Demux57/5 -> Mux64/1
  Demux57/6 -> Mux65/1
  [Ji_1_1] -> Mux60/2
  [Ji_2_2] -> Mux61/2
  [Ji_3_3] -> Mux62/2
  [Ji_2_3] -> Mux63/2
  [Ji_1_3] -> Mux64/2
  [Ji_1_2] -> Mux65/2
  Mux76/1 -> Scope23/1
  Mux77/1 -> Scope23/2
  Mux78/1 -> Scope23/3
  Mux79/1 -> Scope31/1
  Mux80/1 -> Scope31/2
  Mux81/1 -> Scope31/3
  Demux58/1 -> Mux76/1
  Demux58/2 -> Mux77/1
  Demux58/3 -> Mux78/1
  Demux58/4 -> Mux79/1
  Demux58/5 -> Mux80/1
  Demux58/6 -> Mux81/1
  [Ji_1_1] -> Mux76/2
  [Ji_2_2] -> Mux77/2
  [Ji_3_3] -> Mux78/2
  [Ji_2_3] -> Mux79/2
  [Ji_1_3] -> Mux80/2
  [Ji_1_2] -> Mux81/2
  Demux59/6 -> Mux87/1
  [Ji_1_2] -> Mux87/2
  Demux59/3 -> Mux84/1
  [Ji_3_3] -> Mux84/2
  Mux87/1 -> Scope21/3
  [Ji_1_3] -> Mux86/2
  Demux59/4 -> Mux85/1
  depart theta_hat_3/1(y) -> Display11/1, Demux59/1
  Mux85/1 -> Scope21/1
  [Ji_2_2] -> Mux83/2
  Mux84/1 -> Scope20/3
  Mux86/1 -> Scope21/2
  [Ji_2_3] -> Mux85/2
  [Ji_1_1] -> Mux82/2
  Demux59/1 -> Mux82/1
  Demux59/5 -> Mux86/1
  Mux82/1 -> Scope20/1
  Mux83/1 -> Scope20/2
  Demux59/2 -> Mux83/1
  Demux60/6 -> Mux93/1
  [Ji_1_2] -> Mux93/2
  Demux60/3 -> Mux90/1
  [Ji_3_3] -> Mux90/2
  Mux93/1 -> Scope32/3
  [Ji_1_3] -> Mux92/2
  Demux60/4 -> Mux91/1
  depart theta_hat_4/1(y) -> Display14/1, Demux60/1
  Mux91/1 -> Scope32/1
  [Ji_2_2] -> Mux89/2
  Mux90/1 -> Scope24/3
  Mux92/1 -> Scope32/2
  [Ji_2_3] -> Mux91/2
  [Ji_1_1] -> Mux88/2
  Demux60/1 -> Mux88/1
  Demux60/5 -> Mux92/1
  Mux88/1 -> Scope24/1
  Mux89/1 -> Scope24/2
  Demux60/2 -> Mux89/1
  Demux61/6 -> Mux99/1
  [Ji_1_2] -> Mux99/2
  Demux61/3 -> Mux96/1
  [Ji_3_3] -> Mux96/2
  Mux99/1 -> Scope34/3
  [Ji_1_3] -> Mux98/2
  Demux61/4 -> Mux97/1
  Mux97/1 -> Scope34/1
  [Ji_2_2] -> Mux95/2
  Mux96/1 -> Scope33/3
  Mux98/1 -> Scope34/2
  [Ji_2_3] -> Mux97/2
  [Ji_1_1] -> Mux94/2
  Demux61/1 -> Mux94/1
  Demux61/5 -> Mux98/1
  depart theta_hat_5/1(y) -> Demux61/1, Display15/1
  Mux94/1 -> Scope33/1
  Mux95/1 -> Scope33/2
  Demux61/2 -> Mux95/1
  [Ji_1_1] -> Mux100/1
  [Ji_2_2] -> Mux100/2
  [Ji_3_3] -> Mux100/3
  [Ji_2_3] -> Mux100/4
  [Ji_1_3] -> Mux100/5
  [Ji_1_2] -> Mux100/6
  Mux100/1 -> [thetai]
  [tsim] -> process velocity/11(t)
  Constant71/1 -> process velocity/2(T1)
  Step/1 -> leader eta0 Integrator/2
  leader eta0 Integrator/1 -> [eta0], leader ksi0 Integrator/1
  Constant32/1 -> leader control input/2(T1)
  [u0] -> leader eta0 Integrator/1
  Constant130/1 -> process velocity/7(R1)
  [V_init_out] -> leader eta0 Integrator/3
  [u0] -> control input generator agent 5/1(u0)
  [u0] -> control input generator agent 1/1(u0)
  [ui_n_5] -> combine norminal formation control input/5(ui_5)
  [ui_n_3] -> combine norminal formation control input/3(ui_3)
  Constant67/1 -> leader control input/6(Rx2)
  Memory/1 -> [ui_vec]
  [ui_n_4] -> combine norminal formation control input/4(ui_4)
  Clock/1 -> [tsim]
  [u0] -> control input generator agent 3/1(u0)
  control input generator agent 1/1(ui) -> [ui_n_1]
  control input generator agent 2/1(ui) -> [ui_n_2]
  [ui_n_2] -> combine norminal formation control input/2(ui_2)
  [ui_n_1] -> combine norminal formation control input/1(ui_1)
  control input generator agent 4/1(ui) -> [ui_n_4]
  control input generator agent 3/1(ui) -> [ui_n_3]
  [u0] -> control input generator agent 2/1(u0)
  process velocity/1(V_init_out) -> [V_init_out]
  Constant72/1 -> process velocity/4(PZ0)
  Demux1/1 -> ksi_0/1
  Constant64/1 -> leader control input/3(T2)
  Demux1/2 -> ksi_0/2
  combine norminal formation control input/1(ui_vec) -> Memory/1
  Demux22/3 -> eta_0/3
  [tsim] -> leader control input/1(t)
  control input generator agent 5/1(ui) -> [ui_n_5]
  Constant133/1 -> process velocity/9(Ry2)
  Constant70/1 -> process velocity/3(T2)
  leader ksi0 Integrator/1 -> [ksi0]
  Constant134/1 -> process velocity/8(Rx2)
  [u0] -> control input generator agent 4/1(u0)
  Demux1/3 -> ksi_0/3
  Constant132/1 -> process velocity/10(Rz2)
  Demux22/2 -> eta_0/2
  Constant73/1 -> process velocity/5(PZ1)
  Constant66/1 -> leader control input/5(R1)
  Constant68/1 -> leader control input/7(Ry2)
  Demux22/1 -> eta_0/1
  [ksi0] -> Demux1/1
  Constant65/1 -> leader control input/4(R0)
  Constant129/1 -> process velocity/6(R0)
  [eta0] -> Demux22/1
  Constant69/1 -> leader control input/8(Rz2)
  Constant131/1 -> process velocity/1(T0)
  leader control input/1(u0) -> [u0]
  [dw_hat_vec] -> To Workspace9/1
  [zetai_vec] -> To Workspace6/1
  [sgei_vec] -> To Workspace19/1
  [wi_vec] -> To Workspace2/1
  [wci_vec] -> To Workspace/1
  [ksi0] -> To Workspace5/1
  [sgi_vec] -> To Workspace20/1
  [dw_tilt_vec] -> To Workspace10/1
  [dw_vec] -> To Workspace8/1
  [sigma_w_vec] -> To Workspace14/1
  [eta0] -> To Workspace4/1
  [wei_vec] -> To Workspace13/1
  [thetai] -> To Workspace11/1
  [thetai_hat_vec] -> To Workspace7/1
  [V_Phi_Rei_vec] -> To Workspace1/1
  [sigma_bar_w_hat_vec] -> To Workspace12/1
  [u0] -> To Workspace3/1
  [sigma_bar_w_vec] -> To Workspace15/1
  generate angular rate disturbance agent 5/1(dw_5) -> [dw_5]
  [dw_2] -> combine tau1/2(dw_2)
  Constant561/1 -> generate angular rate disturbance agent 2/1(dw_aa_t)
  Constant558/1 -> generate angular rate disturbance agent 1/2(dw_ff_t)
  Constant559/1 -> generate angular rate disturbance agent 1/3(dw_phi_t)
  Constant563/1 -> generate angular rate disturbance agent 2/3(dw_phi_t)
  Constant566/1 -> generate angular rate disturbance agent 3/3(dw_phi_t)
  [tsim] -> generate angular rate disturbance agent 4/4(t)
  [tsim] -> generate angular rate disturbance agent 2/4(t)
  [dw_5] -> combine tau1/5(dw_5)
  Constant562/1 -> generate angular rate disturbance agent 2/2(dw_ff_t)
  [tsim] -> generate angular rate disturbance agent 3/4(t)
  Constant565/1 -> generate angular rate disturbance agent 3/2(dw_ff_t)
  generate angular rate disturbance agent 3/1(dw_3) -> [dw_3]
  Constant572/1 -> generate angular rate disturbance agent 5/2(dw_ff_t)
  [dw_4] -> combine tau1/4(dw_4)
  Constant557/1 -> generate angular rate disturbance agent 1/1(dw_aa_t)
  Constant569/1 -> generate angular rate disturbance agent 4/3(dw_phi_t)
  Constant568/1 -> generate angular rate disturbance agent 4/2(dw_ff_t)
  Constant564/1 -> generate angular rate disturbance agent 3/1(dw_aa_t)
  generate angular rate disturbance agent 4/1(dw_4) -> [dw_4]
  generate angular rate disturbance agent 1/1(dw_1) -> [dw_1]
  Constant573/1 -> generate angular rate disturbance agent 5/3(dw_phi_t)
  [tsim] -> generate angular rate disturbance agent 5/4(t)
  Constant567/1 -> generate angular rate disturbance agent 4/1(dw_aa_t)
  Constant570/1 -> generate angular rate disturbance agent 5/1(dw_aa_t)
  [dw_1] -> combine tau1/1(dw_1)
  [tsim] -> generate angular rate disturbance agent 1/4(t)
  [dw_3] -> combine tau1/3(dw_3)
  generate angular rate disturbance agent 2/1(dw_2) -> [dw_2]
  combine tau1/1(dw_vec) -> [dw_vec]
